simulink library "sm_trackV_lib_chain_track_s46"  (R2026a)
settings: Solver=VariableStepAuto
undefined symbols (not defined in the file): Excv, L1, L10, L11, L12, L13, L14, L15, L16, L17, L18, L19, L2, L20, L21, L22, L23, L24, L25, L26, L27, L28, L29, L3, L30, L31, L32, L33, L34, L35, L36, L37, L38, L39, L4, L40, L41, L42, L43, L44, L45, L46, L5, L6, L7, L8, L9, track_joint_targets
libraries: sm_trackV_lib_chain_segment x184
(part 5 of 5)

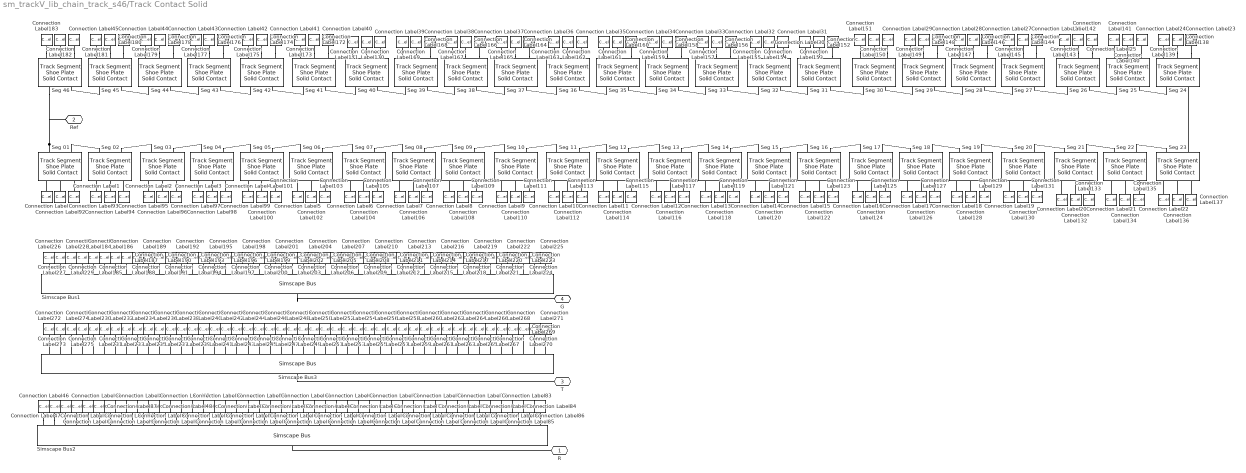
== system sm_trackV_lib_chain_track_s46/Track Contact Solid ==
  Connection Label : ConnectionLabel  Label=R1
  Connection Label1 : ConnectionLabel  Label=R2
  Connection Label10 : ConnectionLabel  Label=R11
  Connection Label100 : ConnectionLabel  Label=G5
  Connection Label101 : ConnectionLabel  Label=T5
  Connection Label102 : ConnectionLabel  Label=G6
  Connection Label103 : ConnectionLabel  Label=T6
  Connection Label104 : ConnectionLabel  Label=G7
  Connection Label105 : ConnectionLabel  Label=T7
  Connection Label106 : ConnectionLabel  Label=G8
  Connection Label107 : ConnectionLabel  Label=T8
  Connection Label108 : ConnectionLabel  Label=G9
  Connection Label109 : ConnectionLabel  Label=T9
  Connection Label11 : ConnectionLabel  Label=R12
  Connection Label110 : ConnectionLabel  Label=G10
  Connection Label111 : ConnectionLabel  Label=T10
  Connection Label112 : ConnectionLabel  Label=G11
  Connection Label113 : ConnectionLabel  Label=T11
  Connection Label114 : ConnectionLabel  Label=G12
  Connection Label115 : ConnectionLabel  Label=T12
  Connection Label116 : ConnectionLabel  Label=G13
  Connection Label117 : ConnectionLabel  Label=T13
  Connection Label118 : ConnectionLabel  Label=G14
  Connection Label119 : ConnectionLabel  Label=T14
  Connection Label12 : ConnectionLabel  Label=R13
  Connection Label120 : ConnectionLabel  Label=G15
  Connection Label121 : ConnectionLabel  Label=T15
  Connection Label122 : ConnectionLabel  Label=G16
  Connection Label123 : ConnectionLabel  Label=T16
  Connection Label124 : ConnectionLabel  Label=G17
  Connection Label125 : ConnectionLabel  Label=T17
  Connection Label126 : ConnectionLabel  Label=G18
  Connection Label127 : ConnectionLabel  Label=T18
  Connection Label128 : ConnectionLabel  Label=G19
  Connection Label129 : ConnectionLabel  Label=T19
  Connection Label13 : ConnectionLabel  Label=R14
  Connection Label130 : ConnectionLabel  Label=G20
  Connection Label131 : ConnectionLabel  Label=T20
  Connection Label132 : ConnectionLabel  Label=G21
  Connection Label133 : ConnectionLabel  Label=T21
  Connection Label134 : ConnectionLabel  Label=G22
  Connection Label135 : ConnectionLabel  Label=T22
  Connection Label136 : ConnectionLabel  Label=G23
  Connection Label137 : ConnectionLabel  Label=T23
  Connection Label138 : ConnectionLabel  Label=G24
  Connection Label139 : ConnectionLabel  Label=T24
  Connection Label14 : ConnectionLabel  Label=R15
  Connection Label140 : ConnectionLabel  Label=G25
  Connection Label141 : ConnectionLabel  Label=T25
  Connection Label142 : ConnectionLabel  Label=G26
  Connection Label143 : ConnectionLabel  Label=T26
  Connection Label144 : ConnectionLabel  Label=G27
  Connection Label145 : ConnectionLabel  Label=T27
  Connection Label146 : ConnectionLabel  Label=G28
  Connection Label147 : ConnectionLabel  Label=T28
  Connection Label148 : ConnectionLabel  Label=G29
  Connection Label149 : ConnectionLabel  Label=T29
  Connection Label15 : ConnectionLabel  Label=R16
  Connection Label150 : ConnectionLabel  Label=G30
  Connection Label151 : ConnectionLabel  Label=T30
  Connection Label152 : ConnectionLabel  Label=G31
  Connection Label153 : ConnectionLabel  Label=T31
  Connection Label154 : ConnectionLabel  Label=G32
  Connection Label155 : ConnectionLabel  Label=T32
  Connection Label156 : ConnectionLabel  Label=G33
  Connection Label157 : ConnectionLabel  Label=T33
  Connection Label158 : ConnectionLabel  Label=G34
  Connection Label159 : ConnectionLabel  Label=T34
  Connection Label16 : ConnectionLabel  Label=R17
  Connection Label160 : ConnectionLabel  Label=G35
  Connection Label161 : ConnectionLabel  Label=T35
  Connection Label162 : ConnectionLabel  Label=G36
  Connection Label163 : ConnectionLabel  Label=T36
  Connection Label164 : ConnectionLabel  Label=G37
  Connection Label165 : ConnectionLabel  Label=T37
  Connection Label166 : ConnectionLabel  Label=G38
  Connection Label167 : ConnectionLabel  Label=T38
  Connection Label168 : ConnectionLabel  Label=G39
  Connection Label169 : ConnectionLabel  Label=T39
  Connection Label17 : ConnectionLabel  Label=R18
  Connection Label170 : ConnectionLabel  Label=G40
  Connection Label171 : ConnectionLabel  Label=T40
  Connection Label172 : ConnectionLabel  Label=G41
  Connection Label173 : ConnectionLabel  Label=T41
  Connection Label174 : ConnectionLabel  Label=G42
  Connection Label175 : ConnectionLabel  Label=T42
  Connection Label176 : ConnectionLabel  Label=G43
  Connection Label177 : ConnectionLabel  Label=T43
  Connection Label178 : ConnectionLabel  Label=G44
  Connection Label179 : ConnectionLabel  Label=T44
  Connection Label18 : ConnectionLabel  Label=R19
  Connection Label180 : ConnectionLabel  Label=G45
  Connection Label181 : ConnectionLabel  Label=T45
  Connection Label182 : ConnectionLabel  Label=G46
  Connection Label183 : ConnectionLabel  Label=T46
  Connection Label184 : ConnectionLabel  Label=G5
  Connection Label185 : ConnectionLabel  Label=G6
  Connection Label186 : ConnectionLabel  Label=G7
  Connection Label187 : ConnectionLabel  Label=G8
  Connection Label188 : ConnectionLabel  Label=G9
  Connection Label189 : ConnectionLabel  Label=G10
  Connection Label19 : ConnectionLabel  Label=R20
  Connection Label190 : ConnectionLabel  Label=G11
  Connection Label191 : ConnectionLabel  Label=G12
  Connection Label192 : ConnectionLabel  Label=G13
  Connection Label193 : ConnectionLabel  Label=G14
  Connection Label194 : ConnectionLabel  Label=G15
  Connection Label195 : ConnectionLabel  Label=G16
  Connection Label196 : ConnectionLabel  Label=G17
  Connection Label197 : ConnectionLabel  Label=G18
  Connection Label198 : ConnectionLabel  Label=G19
  Connection Label199 : ConnectionLabel  Label=G20
  Connection Label2 : ConnectionLabel  Label=R3
  Connection Label20 : ConnectionLabel  Label=R21
  Connection Label200 : ConnectionLabel  Label=G21
  Connection Label201 : ConnectionLabel  Label=G22
  Connection Label202 : ConnectionLabel  Label=G23
  Connection Label203 : ConnectionLabel  Label=G24
  Connection Label204 : ConnectionLabel  Label=G25
  Connection Label205 : ConnectionLabel  Label=G26
  Connection Label206 : ConnectionLabel  Label=G27
  Connection Label207 : ConnectionLabel  Label=G28
  Connection Label208 : ConnectionLabel  Label=G29
  Connection Label209 : ConnectionLabel  Label=G30
  Connection Label21 : ConnectionLabel  Label=R22
  Connection Label210 : ConnectionLabel  Label=G31
  Connection Label211 : ConnectionLabel  Label=G32
  Connection Label212 : ConnectionLabel  Label=G33
  Connection Label213 : ConnectionLabel  Label=G34
  Connection Label214 : ConnectionLabel  Label=G35
  Connection Label215 : ConnectionLabel  Label=G36
  Connection Label216 : ConnectionLabel  Label=G37
  Connection Label217 : ConnectionLabel  Label=G38
  Connection Label218 : ConnectionLabel  Label=G39
  Connection Label219 : ConnectionLabel  Label=G40
  Connection Label22 : ConnectionLabel  Label=R23
  Connection Label220 : ConnectionLabel  Label=G41
  Connection Label221 : ConnectionLabel  Label=G42
  Connection Label222 : ConnectionLabel  Label=G43
  Connection Label223 : ConnectionLabel  Label=G44
  Connection Label224 : ConnectionLabel  Label=G45
  Connection Label225 : ConnectionLabel  Label=G46
  Connection Label226 : ConnectionLabel  Label=G1
  Connection Label227 : ConnectionLabel  Label=G2
  Connection Label228 : ConnectionLabel  Label=G3
  Connection Label229 : ConnectionLabel  Label=G4
  Connection Label23 : ConnectionLabel  Label=R24
  Connection Label230 : ConnectionLabel  Label=T5
  Connection Label231 : ConnectionLabel  Label=T6
  Connection Label232 : ConnectionLabel  Label=T7
  Connection Label233 : ConnectionLabel  Label=T8
  Connection Label234 : ConnectionLabel  Label=T9
  Connection Label235 : ConnectionLabel  Label=T10
  Connection Label236 : ConnectionLabel  Label=T11
  Connection Label237 : ConnectionLabel  Label=T12
  Connection Label238 : ConnectionLabel  Label=T13
  Connection Label239 : ConnectionLabel  Label=T14
  Connection Label24 : ConnectionLabel  Label=R25
  Connection Label240 : ConnectionLabel  Label=T15
  Connection Label241 : ConnectionLabel  Label=T16
  Connection Label242 : ConnectionLabel  Label=T17
  Connection Label243 : ConnectionLabel  Label=T18
  Connection Label244 : ConnectionLabel  Label=T19
  Connection Label245 : ConnectionLabel  Label=T20
  Connection Label246 : ConnectionLabel  Label=T21
  Connection Label247 : ConnectionLabel  Label=T22
  Connection Label248 : ConnectionLabel  Label=T23
  Connection Label249 : ConnectionLabel  Label=T24
  Connection Label25 : ConnectionLabel  Label=R26
  Connection Label250 : ConnectionLabel  Label=T25
  Connection Label251 : ConnectionLabel  Label=T26
  Connection Label252 : ConnectionLabel  Label=T27
  Connection Label253 : ConnectionLabel  Label=T28
  Connection Label254 : ConnectionLabel  Label=T29
  Connection Label255 : ConnectionLabel  Label=T30
  Connection Label256 : ConnectionLabel  Label=T31
  Connection Label257 : ConnectionLabel  Label=T32
  Connection Label258 : ConnectionLabel  Label=T33
  Connection Label259 : ConnectionLabel  Label=T34
  Connection Label26 : ConnectionLabel  Label=R27
  Connection Label260 : ConnectionLabel  Label=T35
  Connection Label261 : ConnectionLabel  Label=T36
  Connection Label262 : ConnectionLabel  Label=T37
  Connection Label263 : ConnectionLabel  Label=T38
  Connection Label264 : ConnectionLabel  Label=T39
  Connection Label265 : ConnectionLabel  Label=T40
  Connection Label266 : ConnectionLabel  Label=T41
  Connection Label267 : ConnectionLabel  Label=T42
  Connection Label268 : ConnectionLabel  Label=T43
  Connection Label269 : ConnectionLabel  Label=T44
  Connection Label27 : ConnectionLabel  Label=R28
  Connection Label270 : ConnectionLabel  Label=T45
  Connection Label271 : ConnectionLabel  Label=T46
  Connection Label272 : ConnectionLabel  Label=T1
  Connection Label273 : ConnectionLabel  Label=T2
  Connection Label274 : ConnectionLabel  Label=T3
  Connection Label275 : ConnectionLabel  Label=T4
  Connection Label28 : ConnectionLabel  Label=R29
  Connection Label29 : ConnectionLabel  Label=R30
  Connection Label3 : ConnectionLabel  Label=R4
  Connection Label30 : ConnectionLabel  Label=R31
  Connection Label31 : ConnectionLabel  Label=R32
  Connection Label32 : ConnectionLabel  Label=R33
  Connection Label33 : ConnectionLabel  Label=R34
  Connection Label34 : ConnectionLabel  Label=R35
  Connection Label35 : ConnectionLabel  Label=R36
  Connection Label36 : ConnectionLabel  Label=R37
  Connection Label37 : ConnectionLabel  Label=R38
  Connection Label38 : ConnectionLabel  Label=R39
  Connection Label39 : ConnectionLabel  Label=R40
  Connection Label4 : ConnectionLabel  Label=R5
  Connection Label40 : ConnectionLabel  Label=R41
  Connection Label41 : ConnectionLabel  Label=R42
  Connection Label42 : ConnectionLabel  Label=R43
  Connection Label43 : ConnectionLabel  Label=R44
  Connection Label44 : ConnectionLabel  Label=R45
  Connection Label45 : ConnectionLabel  Label=R46
  Connection Label46 : ConnectionLabel  Label=R1
  Connection Label47 : ConnectionLabel  Label=R2
  Connection Label48 : ConnectionLabel  Label=R11
  Connection Label49 : ConnectionLabel  Label=R12
  Connection Label5 : ConnectionLabel  Label=R6
  Connection Label50 : ConnectionLabel  Label=R13
  Connection Label51 : ConnectionLabel  Label=R14
  Connection Label52 : ConnectionLabel  Label=R15
  Connection Label53 : ConnectionLabel  Label=R16
  Connection Label54 : ConnectionLabel  Label=R17
  Connection Label55 : ConnectionLabel  Label=R18
  Connection Label56 : ConnectionLabel  Label=R19
  Connection Label57 : ConnectionLabel  Label=R20
  Connection Label58 : ConnectionLabel  Label=R3
  Connection Label59 : ConnectionLabel  Label=R21
  Connection Label6 : ConnectionLabel  Label=R7
  Connection Label60 : ConnectionLabel  Label=R22
  Connection Label61 : ConnectionLabel  Label=R23
  Connection Label62 : ConnectionLabel  Label=R24
  Connection Label63 : ConnectionLabel  Label=R25
  Connection Label64 : ConnectionLabel  Label=R26
  Connection Label65 : ConnectionLabel  Label=R27
  Connection Label66 : ConnectionLabel  Label=R28
  Connection Label67 : ConnectionLabel  Label=R29
  Connection Label68 : ConnectionLabel  Label=R30
  Connection Label69 : ConnectionLabel  Label=R4
  Connection Label7 : ConnectionLabel  Label=R8
  Connection Label70 : ConnectionLabel  Label=R31
  Connection Label71 : ConnectionLabel  Label=R32
  Connection Label72 : ConnectionLabel  Label=R33
  Connection Label73 : ConnectionLabel  Label=R34
  Connection Label74 : ConnectionLabel  Label=R35
  Connection Label75 : ConnectionLabel  Label=R36
  Connection Label76 : ConnectionLabel  Label=R37
  Connection Label77 : ConnectionLabel  Label=R38
  Connection Label78 : ConnectionLabel  Label=R39
  Connection Label79 : ConnectionLabel  Label=R40
  Connection Label8 : ConnectionLabel  Label=R9
  Connection Label80 : ConnectionLabel  Label=R5
  Connection Label81 : ConnectionLabel  Label=R41
  Connection Label82 : ConnectionLabel  Label=R42
  Connection Label83 : ConnectionLabel  Label=R43
  Connection Label84 : ConnectionLabel  Label=R44
  Connection Label85 : ConnectionLabel  Label=R45
  Connection Label86 : ConnectionLabel  Label=R46
  Connection Label87 : ConnectionLabel  Label=R6
  Connection Label88 : ConnectionLabel  Label=R7
  Connection Label89 : ConnectionLabel  Label=R8
  Connection Label9 : ConnectionLabel  Label=R10
  Connection Label90 : ConnectionLabel  Label=R9
  Connection Label91 : ConnectionLabel  Label=R10
  Connection Label92 : ConnectionLabel  Label=G1
  Connection Label93 : ConnectionLabel  Label=T1
  Connection Label94 : ConnectionLabel  Label=G2
  Connection Label95 : ConnectionLabel  Label=T2
  Connection Label96 : ConnectionLabel  Label=G3
  Connection Label97 : ConnectionLabel  Label=T3
  Connection Label98 : ConnectionLabel  Label=G4
  Connection Label99 : ConnectionLabel  Label=T4
  Seg 01 : sm_trackV_lib_chain_segment/Track Segment Shoe Plate Solid Contact  chain_wid=chain_wid  chain_seg_m=chain_seg_m  chain_seg_cg=chain_seg_cg  chain_seg_moi=chain_seg_moi  chain_seg_poi=chain_seg_poi  plate_h=plate_h  plate_xc=plate_xc  plate_thk=plate_thk  pin_sep=pin_sep  plate_ang=plate_ang  plate_clr=plate_clr  plate_opc=plate_opc  pin_len=pin_len  pin_rad=pin_rad  pin_clr=pin_clr  pin_opc=pin_opc  shoe_xc=shoe_xc  shoe_w=shoe_w  shoe_m=shoe_m  shoe_cg=shoe_cg  shoe_moi=shoe_moi  shoe_poi=shoe_poi  shoe_clr=shoe_clr  shoe_opc=shoe_opc  posTgtSpecify=on  posTgtPriority=Low  PositionTargetValue=32.8385  DampingCoefficient=chainDamping  shoe_plate_h=shoe_plate_h  shoe_plate_l=shoe_plate_l  shoe_plate_contact_clr=shoe_plate_contact_clr  shoe_plate_contact_opc=shoe_plate_contact_opc  chain_to_roller_clr=chain_to_roller_clr  chain_to_roller_opc=chain_to_roller_opc  chain_to_teeth_clr=chain_to_teeth_clr  chain_to_teeth_opc=chain_to_teeth_opc
      settings: LibrarySourceBlock=sm_chain_drive_lib/Link Shoe Points
  Seg 02 : sm_trackV_lib_chain_segment/Track Segment Shoe Plate Solid Contact  chain_wid=chain_wid  chain_seg_m=chain_seg_m  chain_seg_cg=chain_seg_cg  chain_seg_moi=chain_seg_moi  chain_seg_poi=chain_seg_poi  plate_h=plate_h  plate_xc=plate_xc  plate_thk=plate_thk  pin_sep=pin_sep  plate_ang=plate_ang  plate_clr=plate_clr  plate_opc=plate_opc  pin_len=pin_len  pin_rad=pin_rad  pin_clr=pin_clr  pin_opc=pin_opc  shoe_xc=shoe_xc  shoe_w=shoe_w  shoe_m=shoe_m  shoe_cg=shoe_cg  shoe_moi=shoe_moi  shoe_poi=shoe_poi  shoe_clr=shoe_clr  shoe_opc=shoe_opc  posTgtSpecify=on  posTgtPriority=Low  PositionTargetValue=32.8407  DampingCoefficient=chainDamping  shoe_plate_h=shoe_plate_h  shoe_plate_l=shoe_plate_l  shoe_plate_contact_clr=shoe_plate_contact_clr  shoe_plate_contact_opc=shoe_plate_contact_opc  chain_to_roller_clr=chain_to_roller_clr  chain_to_roller_opc=chain_to_roller_opc  chain_to_teeth_clr=chain_to_teeth_clr  chain_to_teeth_opc=chain_to_teeth_opc
      settings: LibrarySourceBlock=sm_chain_drive_lib/Tread Segment Shoe Plate Contact
  Seg 03 : sm_trackV_lib_chain_segment/Track Segment Shoe Plate Solid Contact  chain_wid=chain_wid  chain_seg_m=chain_seg_m  chain_seg_cg=chain_seg_cg  chain_seg_moi=chain_seg_moi  chain_seg_poi=chain_seg_poi  plate_h=plate_h  plate_xc=plate_xc  plate_thk=plate_thk  pin_sep=pin_sep  plate_ang=plate_ang  plate_clr=plate_clr  plate_opc=plate_opc  pin_len=pin_len  pin_rad=pin_rad  pin_clr=pin_clr  pin_opc=pin_opc  shoe_xc=shoe_xc  shoe_w=shoe_w  shoe_m=shoe_m  shoe_cg=shoe_cg  shoe_moi=shoe_moi  shoe_poi=shoe_poi  shoe_clr=shoe_clr  shoe_opc=shoe_opc  posTgtSpecify=on  posTgtPriority=Low  PositionTargetValue=32.6576  DampingCoefficient=chainDamping  shoe_plate_h=shoe_plate_h  shoe_plate_l=shoe_plate_l  shoe_plate_contact_clr=shoe_plate_contact_clr  shoe_plate_contact_opc=shoe_plate_contact_opc  chain_to_roller_clr=chain_to_roller_clr  chain_to_roller_opc=chain_to_roller_opc  chain_to_teeth_clr=chain_to_teeth_clr  chain_to_teeth_opc=chain_to_teeth_opc
      settings: LibrarySourceBlock=sm_chain_drive_lib/Tread Segment Shoe Plate Contact
  Seg 04 : sm_trackV_lib_chain_segment/Track Segment Shoe Plate Solid Contact  chain_wid=chain_wid  chain_seg_m=chain_seg_m  chain_seg_cg=chain_seg_cg  chain_seg_moi=chain_seg_moi  chain_seg_poi=chain_seg_poi  plate_h=plate_h  plate_xc=plate_xc  plate_thk=plate_thk  pin_sep=pin_sep  plate_ang=plate_ang  plate_clr=plate_clr  plate_opc=plate_opc  pin_len=pin_len  pin_rad=pin_rad  pin_clr=pin_clr  pin_opc=pin_opc  shoe_xc=shoe_xc  shoe_w=shoe_w  shoe_m=shoe_m  shoe_cg=shoe_cg  shoe_moi=shoe_moi  shoe_poi=shoe_poi  shoe_clr=shoe_clr  shoe_opc=shoe_opc  posTgtSpecify=on  posTgtPriority=Low  PositionTargetValue=5.447  DampingCoefficient=chainDamping  shoe_plate_h=shoe_plate_h  shoe_plate_l=shoe_plate_l  shoe_plate_contact_clr=shoe_plate_contact_clr  shoe_plate_contact_opc=shoe_plate_contact_opc  chain_to_roller_clr=chain_to_roller_clr  chain_to_roller_opc=chain_to_roller_opc  chain_to_teeth_clr=chain_to_teeth_clr  chain_to_teeth_opc=chain_to_teeth_opc
      settings: LibrarySourceBlock=sm_chain_drive_lib/Tread Segment Shoe Plate Contact
  Seg 05 : sm_trackV_lib_chain_segment/Track Segment Shoe Plate Solid Contact  chain_wid=chain_wid  chain_seg_m=chain_seg_m  chain_seg_cg=chain_seg_cg  chain_seg_moi=chain_seg_moi  chain_seg_poi=chain_seg_poi  plate_h=plate_h  plate_xc=plate_xc  plate_thk=plate_thk  pin_sep=pin_sep  plate_ang=plate_ang  plate_clr=plate_clr  plate_opc=plate_opc  pin_len=pin_len  pin_rad=pin_rad  pin_clr=pin_clr  pin_opc=pin_opc  shoe_xc=shoe_xc  shoe_w=shoe_w  shoe_m=shoe_m  shoe_cg=shoe_cg  shoe_moi=shoe_moi  shoe_poi=shoe_poi  shoe_clr=shoe_clr  shoe_opc=shoe_opc  posTgtSpecify=on  posTgtPriority=Low  PositionTargetValue=0.00013277  DampingCoefficient=chainDamping  shoe_plate_h=shoe_plate_h  shoe_plate_l=shoe_plate_l  shoe_plate_contact_clr=shoe_plate_contact_clr  shoe_plate_contact_opc=shoe_plate_contact_opc  chain_to_roller_clr=chain_to_roller_clr  chain_to_roller_opc=chain_to_roller_opc  chain_to_teeth_clr=chain_to_teeth_clr  chain_to_teeth_opc=chain_to_teeth_opc
      settings: LibrarySourceBlock=sm_chain_drive_lib/Tread Segment Shoe Plate Contact
  Seg 06 : sm_trackV_lib_chain_segment/Track Segment Shoe Plate Solid Contact  chain_wid=chain_wid  chain_seg_m=chain_seg_m  chain_seg_cg=chain_seg_cg  chain_seg_moi=chain_seg_moi  chain_seg_poi=chain_seg_poi  plate_h=plate_h  plate_xc=plate_xc  plate_thk=plate_thk  pin_sep=pin_sep  plate_ang=plate_ang  plate_clr=plate_clr  plate_opc=plate_opc  pin_len=pin_len  pin_rad=pin_rad  pin_clr=pin_clr  pin_opc=pin_opc  shoe_xc=shoe_xc  shoe_w=shoe_w  shoe_m=shoe_m  shoe_cg=shoe_cg  shoe_moi=shoe_moi  shoe_poi=shoe_poi  shoe_clr=shoe_clr  shoe_opc=shoe_opc  posTgtSpecify=on  posTgtPriority=Low  PositionTargetValue=1.7589  DampingCoefficient=chainDamping  shoe_plate_h=shoe_plate_h  shoe_plate_l=shoe_plate_l  shoe_plate_contact_clr=shoe_plate_contact_clr  shoe_plate_contact_opc=shoe_plate_contact_opc  chain_to_roller_clr=chain_to_roller_clr  chain_to_roller_opc=chain_to_roller_opc  chain_to_teeth_clr=chain_to_teeth_clr  chain_to_teeth_opc=chain_to_teeth_opc
      settings: LibrarySourceBlock=sm_chain_drive_lib/Tread Segment Shoe Plate Contact
  Seg 07 : sm_trackV_lib_chain_segment/Track Segment Shoe Plate Solid Contact  chain_wid=chain_wid  chain_seg_m=chain_seg_m  chain_seg_cg=chain_seg_cg  chain_seg_moi=chain_seg_moi  chain_seg_poi=chain_seg_poi  plate_h=plate_h  plate_xc=plate_xc  plate_thk=plate_thk  pin_sep=pin_sep  plate_ang=plate_ang  plate_clr=plate_clr  plate_opc=plate_opc  pin_len=pin_len  pin_rad=pin_rad  pin_clr=pin_clr  pin_opc=pin_opc  shoe_xc=shoe_xc  shoe_w=shoe_w  shoe_m=shoe_m  shoe_cg=shoe_cg  shoe_moi=shoe_moi  shoe_poi=shoe_poi  shoe_clr=shoe_clr  shoe_opc=shoe_opc  posTgtSpecify=on  posTgtPriority=Low  PositionTargetValue=0.86753  DampingCoefficient=chainDamping  shoe_plate_h=shoe_plate_h  shoe_plate_l=shoe_plate_l  shoe_plate_contact_clr=shoe_plate_contact_clr  shoe_plate_contact_opc=shoe_plate_contact_opc  chain_to_roller_clr=chain_to_roller_clr  chain_to_roller_opc=chain_to_roller_opc  chain_to_teeth_clr=chain_to_teeth_clr  chain_to_teeth_opc=chain_to_teeth_opc
      settings: LibrarySourceBlock=sm_chain_drive_lib/Tread Segment Shoe Plate Contact
  Seg 08 : sm_trackV_lib_chain_segment/Track Segment Shoe Plate Solid Contact  chain_wid=chain_wid  chain_seg_m=chain_seg_m  chain_seg_cg=chain_seg_cg  chain_seg_moi=chain_seg_moi  chain_seg_poi=chain_seg_poi  plate_h=plate_h  plate_xc=plate_xc  plate_thk=plate_thk  pin_sep=pin_sep  plate_ang=plate_ang  plate_clr=plate_clr  plate_opc=plate_opc  pin_len=pin_len  pin_rad=pin_rad  pin_clr=pin_clr  pin_opc=pin_opc  shoe_xc=shoe_xc  shoe_w=shoe_w  shoe_m=shoe_m  shoe_cg=shoe_cg  shoe_moi=shoe_moi  shoe_poi=shoe_poi  shoe_clr=shoe_clr  shoe_opc=shoe_opc  posTgtSpecify=on  posTgtPriority=Low  PositionTargetValue=-0.00014634  DampingCoefficient=chainDamping  shoe_plate_h=shoe_plate_h  shoe_plate_l=shoe_plate_l  shoe_plate_contact_clr=shoe_plate_contact_clr  shoe_plate_contact_opc=shoe_plate_contact_opc  chain_to_roller_clr=chain_to_roller_clr  chain_to_roller_opc=chain_to_roller_opc  chain_to_teeth_clr=chain_to_teeth_clr  chain_to_teeth_opc=chain_to_teeth_opc
      settings: LibrarySourceBlock=sm_chain_drive_lib/Tread Segment Shoe Plate Contact
  Seg 09 : sm_trackV_lib_chain_segment/Track Segment Shoe Plate Solid Contact  chain_wid=chain_wid  chain_seg_m=chain_seg_m  chain_seg_cg=chain_seg_cg  chain_seg_moi=chain_seg_moi  chain_seg_poi=chain_seg_poi  plate_h=plate_h  plate_xc=plate_xc  plate_thk=plate_thk  pin_sep=pin_sep  plate_ang=plate_ang  plate_clr=plate_clr  plate_opc=plate_opc  pin_len=pin_len  pin_rad=pin_rad  pin_clr=pin_clr  pin_opc=pin_opc  shoe_xc=shoe_xc  shoe_w=shoe_w  shoe_m=shoe_m  shoe_cg=shoe_cg  shoe_moi=shoe_moi  shoe_poi=shoe_poi  shoe_clr=shoe_clr  shoe_opc=shoe_opc  posTgtSpecify=on  posTgtPriority=Low  PositionTargetValue=-0.00033658  DampingCoefficient=chainDamping  shoe_plate_h=shoe_plate_h  shoe_plate_l=shoe_plate_l  shoe_plate_contact_clr=shoe_plate_contact_clr  shoe_plate_contact_opc=shoe_plate_contact_opc  chain_to_roller_clr=chain_to_roller_clr  chain_to_roller_opc=chain_to_roller_opc  chain_to_teeth_clr=chain_to_teeth_clr  chain_to_teeth_opc=chain_to_teeth_opc
      settings: LibrarySourceBlock=sm_chain_drive_lib/Tread Segment Shoe Plate Contact
  Seg 10 : sm_trackV_lib_chain_segment/Track Segment Shoe Plate Solid Contact  chain_wid=chain_wid  chain_seg_m=chain_seg_m  chain_seg_cg=chain_seg_cg  chain_seg_moi=chain_seg_moi  chain_seg_poi=chain_seg_poi  plate_h=plate_h  plate_xc=plate_xc  plate_thk=plate_thk  pin_sep=pin_sep  plate_ang=plate_ang  plate_clr=plate_clr  plate_opc=plate_opc  pin_len=pin_len  pin_rad=pin_rad  pin_clr=pin_clr  pin_opc=pin_opc  shoe_xc=shoe_xc  shoe_w=shoe_w  shoe_m=shoe_m  shoe_cg=shoe_cg  shoe_moi=shoe_moi  shoe_poi=shoe_poi  shoe_clr=shoe_clr  shoe_opc=shoe_opc  posTgtSpecify=on  posTgtPriority=Low  PositionTargetValue=-0.0004294  DampingCoefficient=chainDamping  shoe_plate_h=shoe_plate_h  shoe_plate_l=shoe_plate_l  shoe_plate_contact_clr=shoe_plate_contact_clr  shoe_plate_contact_opc=shoe_plate_contact_opc  chain_to_roller_clr=chain_to_roller_clr  chain_to_roller_opc=chain_to_roller_opc  chain_to_teeth_clr=chain_to_teeth_clr  chain_to_teeth_opc=chain_to_teeth_opc
      settings: LibrarySourceBlock=sm_chain_drive_lib/Tread Segment Shoe Plate Contact
  Seg 11 : sm_trackV_lib_chain_segment/Track Segment Shoe Plate Solid Contact  chain_wid=chain_wid  chain_seg_m=chain_seg_m  chain_seg_cg=chain_seg_cg  chain_seg_moi=chain_seg_moi  chain_seg_poi=chain_seg_poi  plate_h=plate_h  plate_xc=plate_xc  plate_thk=plate_thk  pin_sep=pin_sep  plate_ang=plate_ang  plate_clr=plate_clr  plate_opc=plate_opc  pin_len=pin_len  pin_rad=pin_rad  pin_clr=pin_clr  pin_opc=pin_opc  shoe_xc=shoe_xc  shoe_w=shoe_w  shoe_m=shoe_m  shoe_cg=shoe_cg  shoe_moi=shoe_moi  shoe_poi=shoe_poi  shoe_clr=shoe_clr  shoe_opc=shoe_opc  posTgtSpecify=on  posTgtPriority=Low  PositionTargetValue=-0.00049705  DampingCoefficient=chainDamping  shoe_plate_h=shoe_plate_h  shoe_plate_l=shoe_plate_l  shoe_plate_contact_clr=shoe_plate_contact_clr  shoe_plate_contact_opc=shoe_plate_contact_opc  chain_to_roller_clr=chain_to_roller_clr  chain_to_roller_opc=chain_to_roller_opc  chain_to_teeth_clr=chain_to_teeth_clr  chain_to_teeth_opc=chain_to_teeth_opc
      settings: LibrarySourceBlock=sm_chain_drive_lib/Tread Segment Shoe Plate Contact
  Seg 12 : sm_trackV_lib_chain_segment/Track Segment Shoe Plate Solid Contact  chain_wid=chain_wid  chain_seg_m=chain_seg_m  chain_seg_cg=chain_seg_cg  chain_seg_moi=chain_seg_moi  chain_seg_poi=chain_seg_poi  plate_h=plate_h  plate_xc=plate_xc  plate_thk=plate_thk  pin_sep=pin_sep  plate_ang=plate_ang  plate_clr=plate_clr  plate_opc=plate_opc  pin_len=pin_len  pin_rad=pin_rad  pin_clr=pin_clr  pin_opc=pin_opc  shoe_xc=shoe_xc  shoe_w=shoe_w  shoe_m=shoe_m  shoe_cg=shoe_cg  shoe_moi=shoe_moi  shoe_poi=shoe_poi  shoe_clr=shoe_clr  shoe_opc=shoe_opc  posTgtSpecify=on  posTgtPriority=Low  PositionTargetValue=-0.0005297  DampingCoefficient=chainDamping  shoe_plate_h=shoe_plate_h  shoe_plate_l=shoe_plate_l  shoe_plate_contact_clr=shoe_plate_contact_clr  shoe_plate_contact_opc=shoe_plate_contact_opc  chain_to_roller_clr=chain_to_roller_clr  chain_to_roller_opc=chain_to_roller_opc  chain_to_teeth_clr=chain_to_teeth_clr  chain_to_teeth_opc=chain_to_teeth_opc
      settings: LibrarySourceBlock=sm_chain_drive_lib/Tread Segment Shoe Plate Contact
  Seg 13 : sm_trackV_lib_chain_segment/Track Segment Shoe Plate Solid Contact  chain_wid=chain_wid  chain_seg_m=chain_seg_m  chain_seg_cg=chain_seg_cg  chain_seg_moi=chain_seg_moi  chain_seg_poi=chain_seg_poi  plate_h=plate_h  plate_xc=plate_xc  plate_thk=plate_thk  pin_sep=pin_sep  plate_ang=plate_ang  plate_clr=plate_clr  plate_opc=plate_opc  pin_len=pin_len  pin_rad=pin_rad  pin_clr=pin_clr  pin_opc=pin_opc  shoe_xc=shoe_xc  shoe_w=shoe_w  shoe_m=shoe_m  shoe_cg=shoe_cg  shoe_moi=shoe_moi  shoe_poi=shoe_poi  shoe_clr=shoe_clr  shoe_opc=shoe_opc  posTgtSpecify=on  posTgtPriority=Low  PositionTargetValue=-0.00052132  DampingCoefficient=chainDamping  shoe_plate_h=shoe_plate_h  shoe_plate_l=shoe_plate_l  shoe_plate_contact_clr=shoe_plate_contact_clr  shoe_plate_contact_opc=shoe_plate_contact_opc  chain_to_roller_clr=chain_to_roller_clr  chain_to_roller_opc=chain_to_roller_opc  chain_to_teeth_clr=chain_to_teeth_clr  chain_to_teeth_opc=chain_to_teeth_opc
      settings: LibrarySourceBlock=sm_chain_drive_lib/Tread Segment Shoe Plate Contact
  Seg 14 : sm_trackV_lib_chain_segment/Track Segment Shoe Plate Solid Contact  chain_wid=chain_wid  chain_seg_m=chain_seg_m  chain_seg_cg=chain_seg_cg  chain_seg_moi=chain_seg_moi  chain_seg_poi=chain_seg_poi  plate_h=plate_h  plate_xc=plate_xc  plate_thk=plate_thk  pin_sep=pin_sep  plate_ang=plate_ang  plate_clr=plate_clr  plate_opc=plate_opc  pin_len=pin_len  pin_rad=pin_rad  pin_clr=pin_clr  pin_opc=pin_opc  shoe_xc=shoe_xc  shoe_w=shoe_w  shoe_m=shoe_m  shoe_cg=shoe_cg  shoe_moi=shoe_moi  shoe_poi=shoe_poi  shoe_clr=shoe_clr  shoe_opc=shoe_opc  posTgtSpecify=on  posTgtPriority=Low  PositionTargetValue=-0.00046966  DampingCoefficient=chainDamping  shoe_plate_h=shoe_plate_h  shoe_plate_l=shoe_plate_l  shoe_plate_contact_clr=shoe_plate_contact_clr  shoe_plate_contact_opc=shoe_plate_contact_opc  chain_to_roller_clr=chain_to_roller_clr  chain_to_roller_opc=chain_to_roller_opc  chain_to_teeth_clr=chain_to_teeth_clr  chain_to_teeth_opc=chain_to_teeth_opc
      settings: LibrarySourceBlock=sm_chain_drive_lib/Tread Segment Shoe Plate Contact
  Seg 15 : sm_trackV_lib_chain_segment/Track Segment Shoe Plate Solid Contact  chain_wid=chain_wid  chain_seg_m=chain_seg_m  chain_seg_cg=chain_seg_cg  chain_seg_moi=chain_seg_moi  chain_seg_poi=chain_seg_poi  plate_h=plate_h  plate_xc=plate_xc  plate_thk=plate_thk  pin_sep=pin_sep  plate_ang=plate_ang  plate_clr=plate_clr  plate_opc=plate_opc  pin_len=pin_len  pin_rad=pin_rad  pin_clr=pin_clr  pin_opc=pin_opc  shoe_xc=shoe_xc  shoe_w=shoe_w  shoe_m=shoe_m  shoe_cg=shoe_cg  shoe_moi=shoe_moi  shoe_poi=shoe_poi  shoe_clr=shoe_clr  shoe_opc=shoe_opc  posTgtSpecify=on  posTgtPriority=Low  PositionTargetValue=-0.00038011  DampingCoefficient=chainDamping  shoe_plate_h=shoe_plate_h  shoe_plate_l=shoe_plate_l  shoe_plate_contact_clr=shoe_plate_contact_clr  shoe_plate_contact_opc=shoe_plate_contact_opc  chain_to_roller_clr=chain_to_roller_clr  chain_to_roller_opc=chain_to_roller_opc  chain_to_teeth_clr=chain_to_teeth_clr  chain_to_teeth_opc=chain_to_teeth_opc
      settings: LibrarySourceBlock=sm_chain_drive_lib/Tread Segment Shoe Plate Contact
  Seg 16 : sm_trackV_lib_chain_segment/Track Segment Shoe Plate Solid Contact  chain_wid=chain_wid  chain_seg_m=chain_seg_m  chain_seg_cg=chain_seg_cg  chain_seg_moi=chain_seg_moi  chain_seg_poi=chain_seg_poi  plate_h=plate_h  plate_xc=plate_xc  plate_thk=plate_thk  pin_sep=pin_sep  plate_ang=plate_ang  plate_clr=plate_clr  plate_opc=plate_opc  pin_len=pin_len  pin_rad=pin_rad  pin_clr=pin_clr  pin_opc=pin_opc  shoe_xc=shoe_xc  shoe_w=shoe_w  shoe_m=shoe_m  shoe_cg=shoe_cg  shoe_moi=shoe_moi  shoe_poi=shoe_poi  shoe_clr=shoe_clr  shoe_opc=shoe_opc  posTgtSpecify=on  posTgtPriority=Low  PositionTargetValue=-0.00026621  DampingCoefficient=chainDamping  shoe_plate_h=shoe_plate_h  shoe_plate_l=shoe_plate_l  shoe_plate_contact_clr=shoe_plate_contact_clr  shoe_plate_contact_opc=shoe_plate_contact_opc  chain_to_roller_clr=chain_to_roller_clr  chain_to_roller_opc=chain_to_roller_opc  chain_to_teeth_clr=chain_to_teeth_clr  chain_to_teeth_opc=chain_to_teeth_opc
      settings: LibrarySourceBlock=sm_chain_drive_lib/Tread Segment Shoe Plate Contact
  Seg 17 : sm_trackV_lib_chain_segment/Track Segment Shoe Plate Solid Contact  chain_wid=chain_wid  chain_seg_m=chain_seg_m  chain_seg_cg=chain_seg_cg  chain_seg_moi=chain_seg_moi  chain_seg_poi=chain_seg_poi  plate_h=plate_h  plate_xc=plate_xc  plate_thk=plate_thk  pin_sep=pin_sep  plate_ang=plate_ang  plate_clr=plate_clr  plate_opc=plate_opc  pin_len=pin_len  pin_rad=pin_rad  pin_clr=pin_clr  pin_opc=pin_opc  shoe_xc=shoe_xc  shoe_w=shoe_w  shoe_m=shoe_m  shoe_cg=shoe_cg  shoe_moi=shoe_moi  shoe_poi=shoe_poi  shoe_clr=shoe_clr  shoe_opc=shoe_opc  posTgtSpecify=on  posTgtPriority=Low  PositionTargetValue=4.6763e-05  DampingCoefficient=chainDamping  shoe_plate_h=shoe_plate_h  shoe_plate_l=shoe_plate_l  shoe_plate_contact_clr=shoe_plate_contact_clr  shoe_plate_contact_opc=shoe_plate_contact_opc  chain_to_roller_clr=chain_to_roller_clr  chain_to_roller_opc=chain_to_roller_opc  chain_to_teeth_clr=chain_to_teeth_clr  chain_to_teeth_opc=chain_to_teeth_opc
      settings: LibrarySourceBlock=sm_chain_drive_lib/Tread Segment Shoe Plate Contact
  Seg 18 : sm_trackV_lib_chain_segment/Track Segment Shoe Plate Solid Contact  chain_wid=chain_wid  chain_seg_m=chain_seg_m  chain_seg_cg=chain_seg_cg  chain_seg_moi=chain_seg_moi  chain_seg_poi=chain_seg_poi  plate_h=plate_h  plate_xc=plate_xc  plate_thk=plate_thk  pin_sep=pin_sep  plate_ang=plate_ang  plate_clr=plate_clr  plate_opc=plate_opc  pin_len=pin_len  pin_rad=pin_rad  pin_clr=pin_clr  pin_opc=pin_opc  shoe_xc=shoe_xc  shoe_w=shoe_w  shoe_m=shoe_m  shoe_cg=shoe_cg  shoe_moi=shoe_moi  shoe_poi=shoe_poi  shoe_clr=shoe_clr  shoe_opc=shoe_opc  posTgtSpecify=on  posTgtPriority=Low  PositionTargetValue=1.1075  DampingCoefficient=chainDamping  shoe_plate_h=shoe_plate_h  shoe_plate_l=shoe_plate_l  shoe_plate_contact_clr=shoe_plate_contact_clr  shoe_plate_contact_opc=shoe_plate_contact_opc  chain_to_roller_clr=chain_to_roller_clr  chain_to_roller_opc=chain_to_roller_opc  chain_to_teeth_clr=chain_to_teeth_clr  chain_to_teeth_opc=chain_to_teeth_opc
      settings: LibrarySourceBlock=sm_chain_drive_lib/Tread Segment Shoe Plate Contact
  Seg 19 : sm_trackV_lib_chain_segment/Track Segment Shoe Plate Solid Contact  chain_wid=chain_wid  chain_seg_m=chain_seg_m  chain_seg_cg=chain_seg_cg  chain_seg_moi=chain_seg_moi  chain_seg_poi=chain_seg_poi  plate_h=plate_h  plate_xc=plate_xc  plate_thk=plate_thk  pin_sep=pin_sep  plate_ang=plate_ang  plate_clr=plate_clr  plate_opc=plate_opc  pin_len=pin_len  pin_rad=pin_rad  pin_clr=pin_clr  pin_opc=pin_opc  shoe_xc=shoe_xc  shoe_w=shoe_w  shoe_m=shoe_m  shoe_cg=shoe_cg  shoe_moi=shoe_moi  shoe_poi=shoe_poi  shoe_clr=shoe_clr  shoe_opc=shoe_opc  posTgtSpecify=on  posTgtPriority=Low  PositionTargetValue=0.12453  DampingCoefficient=chainDamping  shoe_plate_h=shoe_plate_h  shoe_plate_l=shoe_plate_l  shoe_plate_contact_clr=shoe_plate_contact_clr  shoe_plate_contact_opc=shoe_plate_contact_opc  chain_to_roller_clr=chain_to_roller_clr  chain_to_roller_opc=chain_to_roller_opc  chain_to_teeth_clr=chain_to_teeth_clr  chain_to_teeth_opc=chain_to_teeth_opc
      settings: LibrarySourceBlock=sm_chain_drive_lib/Tread Segment Shoe Plate Contact
  Seg 20 : sm_trackV_lib_chain_segment/Track Segment Shoe Plate Solid Contact  chain_wid=chain_wid  chain_seg_m=chain_seg_m  chain_seg_cg=chain_seg_cg  chain_seg_moi=chain_seg_moi  chain_seg_poi=chain_seg_poi  plate_h=plate_h  plate_xc=plate_xc  plate_thk=plate_thk  pin_sep=pin_sep  plate_ang=plate_ang  plate_clr=plate_clr  plate_opc=plate_opc  pin_len=pin_len  pin_rad=pin_rad  pin_clr=pin_clr  pin_opc=pin_opc  shoe_xc=shoe_xc  shoe_w=shoe_w  shoe_m=shoe_m  shoe_cg=shoe_cg  shoe_moi=shoe_moi  shoe_poi=shoe_poi  shoe_clr=shoe_clr  shoe_opc=shoe_opc  posTgtSpecify=on  posTgtPriority=Low  PositionTargetValue=6.4867e-05  DampingCoefficient=chainDamping  shoe_plate_h=shoe_plate_h  shoe_plate_l=shoe_plate_l  shoe_plate_contact_clr=shoe_plate_contact_clr  shoe_plate_contact_opc=shoe_plate_contact_opc  chain_to_roller_clr=chain_to_roller_clr  chain_to_roller_opc=chain_to_roller_opc  chain_to_teeth_clr=chain_to_teeth_clr  chain_to_teeth_opc=chain_to_teeth_opc
      settings: LibrarySourceBlock=sm_chain_drive_lib/Tread Segment Shoe Plate Contact
  Seg 21 : sm_trackV_lib_chain_segment/Track Segment Shoe Plate Solid Contact  chain_wid=chain_wid  chain_seg_m=chain_seg_m  chain_seg_cg=chain_seg_cg  chain_seg_moi=chain_seg_moi  chain_seg_poi=chain_seg_poi  plate_h=plate_h  plate_xc=plate_xc  plate_thk=plate_thk  pin_sep=pin_sep  plate_ang=plate_ang  plate_clr=plate_clr  plate_opc=plate_opc  pin_len=pin_len  pin_rad=pin_rad  pin_clr=pin_clr  pin_opc=pin_opc  shoe_xc=shoe_xc  shoe_w=shoe_w  shoe_m=shoe_m  shoe_cg=shoe_cg  shoe_moi=shoe_moi  shoe_poi=shoe_poi  shoe_clr=shoe_clr  shoe_opc=shoe_opc  posTgtSpecify=on  posTgtPriority=Low  PositionTargetValue=11.1152  DampingCoefficient=chainDamping  shoe_plate_h=shoe_plate_h  shoe_plate_l=shoe_plate_l  shoe_plate_contact_clr=shoe_plate_contact_clr  shoe_plate_contact_opc=shoe_plate_contact_opc  chain_to_roller_clr=chain_to_roller_clr  chain_to_roller_opc=chain_to_roller_opc  chain_to_teeth_clr=chain_to_teeth_clr  chain_to_teeth_opc=chain_to_teeth_opc
      settings: LibrarySourceBlock=sm_chain_drive_lib/Tread Segment Shoe Plate Contact
  Seg 22 : sm_trackV_lib_chain_segment/Track Segment Shoe Plate Solid Contact  chain_wid=chain_wid  chain_seg_m=chain_seg_m  chain_seg_cg=chain_seg_cg  chain_seg_moi=chain_seg_moi  chain_seg_poi=chain_seg_poi  plate_h=plate_h  plate_xc=plate_xc  plate_thk=plate_thk  pin_sep=pin_sep  plate_ang=plate_ang  plate_clr=plate_clr  plate_opc=plate_opc  pin_len=pin_len  pin_rad=pin_rad  pin_clr=pin_clr  pin_opc=pin_opc  shoe_xc=shoe_xc  shoe_w=shoe_w  shoe_m=shoe_m  shoe_cg=shoe_cg  shoe_moi=shoe_moi  shoe_poi=shoe_poi  shoe_clr=shoe_clr  shoe_opc=shoe_opc  posTgtSpecify=on  posTgtPriority=Low  PositionTargetValue=30.3431  DampingCoefficient=chainDamping  shoe_plate_h=shoe_plate_h  shoe_plate_l=shoe_plate_l  shoe_plate_contact_clr=shoe_plate_contact_clr  shoe_plate_contact_opc=shoe_plate_contact_opc  chain_to_roller_clr=chain_to_roller_clr  chain_to_roller_opc=chain_to_roller_opc  chain_to_teeth_clr=chain_to_teeth_clr  chain_to_teeth_opc=chain_to_teeth_opc
      settings: LibrarySourceBlock=sm_chain_drive_lib/Tread Segment Shoe Plate Contact
  Seg 23 : sm_trackV_lib_chain_segment/Track Segment Shoe Plate Solid Contact  chain_wid=chain_wid  chain_seg_m=chain_seg_m  chain_seg_cg=chain_seg_cg  chain_seg_moi=chain_seg_moi  chain_seg_poi=chain_seg_poi  plate_h=plate_h  plate_xc=plate_xc  plate_thk=plate_thk  pin_sep=pin_sep  plate_ang=plate_ang  plate_clr=plate_clr  plate_opc=plate_opc  pin_len=pin_len  pin_rad=pin_rad  pin_clr=pin_clr  pin_opc=pin_opc  shoe_xc=shoe_xc  shoe_w=shoe_w  shoe_m=shoe_m  shoe_cg=shoe_cg  shoe_moi=shoe_moi  shoe_poi=shoe_poi  shoe_clr=shoe_clr  shoe_opc=shoe_opc  posTgtSpecify=on  posTgtPriority=Low  PositionTargetValue=32.3566  DampingCoefficient=chainDamping  shoe_plate_h=shoe_plate_h  shoe_plate_l=shoe_plate_l  shoe_plate_contact_clr=shoe_plate_contact_clr  shoe_plate_contact_opc=shoe_plate_contact_opc  chain_to_roller_clr=chain_to_roller_clr  chain_to_roller_opc=chain_to_roller_opc  chain_to_teeth_clr=chain_to_teeth_clr  chain_to_teeth_opc=chain_to_teeth_opc
      settings: LibrarySourceBlock=sm_chain_drive_lib/Tread Segment Shoe Plate Contact
  Seg 24 : sm_trackV_lib_chain_segment/Track Segment Shoe Plate Solid Contact  chain_wid=chain_wid  chain_seg_m=chain_seg_m  chain_seg_cg=chain_seg_cg  chain_seg_moi=chain_seg_moi  chain_seg_poi=chain_seg_poi  plate_h=plate_h  plate_xc=plate_xc  plate_thk=plate_thk  pin_sep=pin_sep  plate_ang=plate_ang  plate_clr=plate_clr  plate_opc=plate_opc  pin_len=pin_len  pin_rad=pin_rad  pin_clr=pin_clr  pin_opc=pin_opc  shoe_xc=shoe_xc  shoe_w=shoe_w  shoe_m=shoe_m  shoe_cg=shoe_cg  shoe_moi=shoe_moi  shoe_poi=shoe_poi  shoe_clr=shoe_clr  shoe_opc=shoe_opc  posTgtSpecify=on  posTgtPriority=Low  PositionTargetValue=31.2315  DampingCoefficient=chainDamping  shoe_plate_h=shoe_plate_h  shoe_plate_l=shoe_plate_l  shoe_plate_contact_clr=shoe_plate_contact_clr  shoe_plate_contact_opc=shoe_plate_contact_opc  chain_to_roller_clr=chain_to_roller_clr  chain_to_roller_opc=chain_to_roller_opc  chain_to_teeth_clr=chain_to_teeth_clr  chain_to_teeth_opc=chain_to_teeth_opc
      settings: LibrarySourceBlock=sm_chain_drive_lib/Tread Segment Shoe Plate Contact
  Seg 25 : sm_trackV_lib_chain_segment/Track Segment Shoe Plate Solid Contact  chain_wid=chain_wid  chain_seg_m=chain_seg_m  chain_seg_cg=chain_seg_cg  chain_seg_moi=chain_seg_moi  chain_seg_poi=chain_seg_poi  plate_h=plate_h  plate_xc=plate_xc  plate_thk=plate_thk  pin_sep=pin_sep  plate_ang=plate_ang  plate_clr=plate_clr  plate_opc=plate_opc  pin_len=pin_len  pin_rad=pin_rad  pin_clr=pin_clr  pin_opc=pin_opc  shoe_xc=shoe_xc  shoe_w=shoe_w  shoe_m=shoe_m  shoe_cg=shoe_cg  shoe_moi=shoe_moi  shoe_poi=shoe_poi  shoe_clr=shoe_clr  shoe_opc=shoe_opc  posTgtSpecify=on  posTgtPriority=Low  PositionTargetValue=32.7074  DampingCoefficient=chainDamping  shoe_plate_h=shoe_plate_h  shoe_plate_l=shoe_plate_l  shoe_plate_contact_clr=shoe_plate_contact_clr  shoe_plate_contact_opc=shoe_plate_contact_opc  chain_to_roller_clr=chain_to_roller_clr  chain_to_roller_opc=chain_to_roller_opc  chain_to_teeth_clr=chain_to_teeth_clr  chain_to_teeth_opc=chain_to_teeth_opc
      settings: LibrarySourceBlock=sm_chain_drive_lib/Tread Segment Shoe Plate Contact
  Seg 26 : sm_trackV_lib_chain_segment/Track Segment Shoe Plate Solid Contact  chain_wid=chain_wid  chain_seg_m=chain_seg_m  chain_seg_cg=chain_seg_cg  chain_seg_moi=chain_seg_moi  chain_seg_poi=chain_seg_poi  plate_h=plate_h  plate_xc=plate_xc  plate_thk=plate_thk  pin_sep=pin_sep  plate_ang=plate_ang  plate_clr=plate_clr  plate_opc=plate_opc  pin_len=pin_len  pin_rad=pin_rad  pin_clr=pin_clr  pin_opc=pin_opc  shoe_xc=shoe_xc  shoe_w=shoe_w  shoe_m=shoe_m  shoe_cg=shoe_cg  shoe_moi=shoe_moi  shoe_poi=shoe_poi  shoe_clr=shoe_clr  shoe_opc=shoe_opc  posTgtSpecify=on  posTgtPriority=Low  PositionTargetValue=29.2112  DampingCoefficient=chainDamping  shoe_plate_h=shoe_plate_h  shoe_plate_l=shoe_plate_l  shoe_plate_contact_clr=shoe_plate_contact_clr  shoe_plate_contact_opc=shoe_plate_contact_opc  chain_to_roller_clr=chain_to_roller_clr  chain_to_roller_opc=chain_to_roller_opc  chain_to_teeth_clr=chain_to_teeth_clr  chain_to_teeth_opc=chain_to_teeth_opc
      settings: LibrarySourceBlock=sm_chain_drive_lib/Tread Segment Shoe Plate Contact
  Seg 27 : sm_trackV_lib_chain_segment/Track Segment Shoe Plate Solid Contact  chain_wid=chain_wid  chain_seg_m=chain_seg_m  chain_seg_cg=chain_seg_cg  chain_seg_moi=chain_seg_moi  chain_seg_poi=chain_seg_poi  plate_h=plate_h  plate_xc=plate_xc  plate_thk=plate_thk  pin_sep=pin_sep  plate_ang=plate_ang  plate_clr=plate_clr  plate_opc=plate_opc  pin_len=pin_len  pin_rad=pin_rad  pin_clr=pin_clr  pin_opc=pin_opc  shoe_xc=shoe_xc  shoe_w=shoe_w  shoe_m=shoe_m  shoe_cg=shoe_cg  shoe_moi=shoe_moi  shoe_poi=shoe_poi  shoe_clr=shoe_clr  shoe_opc=shoe_opc  posTgtSpecify=on  posTgtPriority=Low  PositionTargetValue=7.6812  DampingCoefficient=chainDamping  shoe_plate_h=shoe_plate_h  shoe_plate_l=shoe_plate_l  shoe_plate_contact_clr=shoe_plate_contact_clr  shoe_plate_contact_opc=shoe_plate_contact_opc  chain_to_roller_clr=chain_to_roller_clr  chain_to_roller_opc=chain_to_roller_opc  chain_to_teeth_clr=chain_to_teeth_clr  chain_to_teeth_opc=chain_to_teeth_opc
      settings: LibrarySourceBlock=sm_chain_drive_lib/Tread Segment Shoe Plate Contact
  Seg 28 : sm_trackV_lib_chain_segment/Track Segment Shoe Plate Solid Contact  chain_wid=chain_wid  chain_seg_m=chain_seg_m  chain_seg_cg=chain_seg_cg  chain_seg_moi=chain_seg_moi  chain_seg_poi=chain_seg_poi  plate_h=plate_h  plate_xc=plate_xc  plate_thk=plate_thk  pin_sep=pin_sep  plate_ang=plate_ang  plate_clr=plate_clr  plate_opc=plate_opc  pin_len=pin_len  pin_rad=pin_rad  pin_clr=pin_clr  pin_opc=pin_opc  shoe_xc=shoe_xc  shoe_w=shoe_w  shoe_m=shoe_m  shoe_cg=shoe_cg  shoe_moi=shoe_moi  shoe_poi=shoe_poi  shoe_clr=shoe_clr  shoe_opc=shoe_opc  posTgtSpecify=on  posTgtPriority=Low  PositionTargetValue=-3.9493e-05  DampingCoefficient=chainDamping  shoe_plate_h=shoe_plate_h  shoe_plate_l=shoe_plate_l  shoe_plate_contact_clr=shoe_plate_contact_clr  shoe_plate_contact_opc=shoe_plate_contact_opc  chain_to_roller_clr=chain_to_roller_clr  chain_to_roller_opc=chain_to_roller_opc  chain_to_teeth_clr=chain_to_teeth_clr  chain_to_teeth_opc=chain_to_teeth_opc
      settings: LibrarySourceBlock=sm_chain_drive_lib/Tread Segment Shoe Plate Contact
  Seg 29 : sm_trackV_lib_chain_segment/Track Segment Shoe Plate Solid Contact  chain_wid=chain_wid  chain_seg_m=chain_seg_m  chain_seg_cg=chain_seg_cg  chain_seg_moi=chain_seg_moi  chain_seg_poi=chain_seg_poi  plate_h=plate_h  plate_xc=plate_xc  plate_thk=plate_thk  pin_sep=pin_sep  plate_ang=plate_ang  plate_clr=plate_clr  plate_opc=plate_opc  pin_len=pin_len  pin_rad=pin_rad  pin_clr=pin_clr  pin_opc=pin_opc  shoe_xc=shoe_xc  shoe_w=shoe_w  shoe_m=shoe_m  shoe_cg=shoe_cg  shoe_moi=shoe_moi  shoe_poi=shoe_poi  shoe_clr=shoe_clr  shoe_opc=shoe_opc  posTgtSpecify=on  posTgtPriority=Low  PositionTargetValue=-4.2189e-05  DampingCoefficient=chainDamping  shoe_plate_h=shoe_plate_h  shoe_plate_l=shoe_plate_l  shoe_plate_contact_clr=shoe_plate_contact_clr  shoe_plate_contact_opc=shoe_plate_contact_opc  chain_to_roller_clr=chain_to_roller_clr  chain_to_roller_opc=chain_to_roller_opc  chain_to_teeth_clr=chain_to_teeth_clr  chain_to_teeth_opc=chain_to_teeth_opc
      settings: LibrarySourceBlock=sm_chain_drive_lib/Tread Segment Shoe Plate Contact
  Seg 30 : sm_trackV_lib_chain_segment/Track Segment Shoe Plate Solid Contact  chain_wid=chain_wid  chain_seg_m=chain_seg_m  chain_seg_cg=chain_seg_cg  chain_seg_moi=chain_seg_moi  chain_seg_poi=chain_seg_poi  plate_h=plate_h  plate_xc=plate_xc  plate_thk=plate_thk  pin_sep=pin_sep  plate_ang=plate_ang  plate_clr=plate_clr  plate_opc=plate_opc  pin_len=pin_len  pin_rad=pin_rad  pin_clr=pin_clr  pin_opc=pin_opc  shoe_xc=shoe_xc  shoe_w=shoe_w  shoe_m=shoe_m  shoe_cg=shoe_cg  shoe_moi=shoe_moi  shoe_poi=shoe_poi  shoe_clr=shoe_clr  shoe_opc=shoe_opc  posTgtSpecify=on  posTgtPriority=Low  PositionTargetValue=-3.4821e-05  DampingCoefficient=chainDamping  shoe_plate_h=shoe_plate_h  shoe_plate_l=shoe_plate_l  shoe_plate_contact_clr=shoe_plate_contact_clr  shoe_plate_contact_opc=shoe_plate_contact_opc  chain_to_roller_clr=chain_to_roller_clr  chain_to_roller_opc=chain_to_roller_opc  chain_to_teeth_clr=chain_to_teeth_clr  chain_to_teeth_opc=chain_to_teeth_opc
      settings: LibrarySourceBlock=sm_chain_drive_lib/Tread Segment Shoe Plate Contact
  Seg 31 : sm_trackV_lib_chain_segment/Track Segment Shoe Plate Solid Contact  chain_wid=chain_wid  chain_seg_m=chain_seg_m  chain_seg_cg=chain_seg_cg  chain_seg_moi=chain_seg_moi  chain_seg_poi=chain_seg_poi  plate_h=plate_h  plate_xc=plate_xc  plate_thk=plate_thk  pin_sep=pin_sep  plate_ang=plate_ang  plate_clr=plate_clr  plate_opc=plate_opc  pin_len=pin_len  pin_rad=pin_rad  pin_clr=pin_clr  pin_opc=pin_opc  shoe_xc=shoe_xc  shoe_w=shoe_w  shoe_m=shoe_m  shoe_cg=shoe_cg  shoe_moi=shoe_moi  shoe_poi=shoe_poi  shoe_clr=shoe_clr  shoe_opc=shoe_opc  posTgtSpecify=on  posTgtPriority=Low  PositionTargetValue=-3.2281e-05  DampingCoefficient=chainDamping  shoe_plate_h=shoe_plate_h  shoe_plate_l=shoe_plate_l  shoe_plate_contact_clr=shoe_plate_contact_clr  shoe_plate_contact_opc=shoe_plate_contact_opc  chain_to_roller_clr=chain_to_roller_clr  chain_to_roller_opc=chain_to_roller_opc  chain_to_teeth_clr=chain_to_teeth_clr  chain_to_teeth_opc=chain_to_teeth_opc
      settings: LibrarySourceBlock=sm_chain_drive_lib/Tread Segment Shoe Plate Contact
  Seg 32 : sm_trackV_lib_chain_segment/Track Segment Shoe Plate Solid Contact  chain_wid=chain_wid  chain_seg_m=chain_seg_m  chain_seg_cg=chain_seg_cg  chain_seg_moi=chain_seg_moi  chain_seg_poi=chain_seg_poi  plate_h=plate_h  plate_xc=plate_xc  plate_thk=plate_thk  pin_sep=pin_sep  plate_ang=plate_ang  plate_clr=plate_clr  plate_opc=plate_opc  pin_len=pin_len  pin_rad=pin_rad  pin_clr=pin_clr  pin_opc=pin_opc  shoe_xc=shoe_xc  shoe_w=shoe_w  shoe_m=shoe_m  shoe_cg=shoe_cg  shoe_moi=shoe_moi  shoe_poi=shoe_poi  shoe_clr=shoe_clr  shoe_opc=shoe_opc  posTgtSpecify=on  posTgtPriority=Low  PositionTargetValue=-2.2438e-05  DampingCoefficient=chainDamping  shoe_plate_h=shoe_plate_h  shoe_plate_l=shoe_plate_l  shoe_plate_contact_clr=shoe_plate_contact_clr  shoe_plate_contact_opc=shoe_plate_contact_opc  chain_to_roller_clr=chain_to_roller_clr  chain_to_roller_opc=chain_to_roller_opc  chain_to_teeth_clr=chain_to_teeth_clr  chain_to_teeth_opc=chain_to_teeth_opc
      settings: LibrarySourceBlock=sm_chain_drive_lib/Tread Segment Shoe Plate Contact
  Seg 33 : sm_trackV_lib_chain_segment/Track Segment Shoe Plate Solid Contact  chain_wid=chain_wid  chain_seg_m=chain_seg_m  chain_seg_cg=chain_seg_cg  chain_seg_moi=chain_seg_moi  chain_seg_poi=chain_seg_poi  plate_h=plate_h  plate_xc=plate_xc  plate_thk=plate_thk  pin_sep=pin_sep  plate_ang=plate_ang  plate_clr=plate_clr  plate_opc=plate_opc  pin_len=pin_len  pin_rad=pin_rad  pin_clr=pin_clr  pin_opc=pin_opc  shoe_xc=shoe_xc  shoe_w=shoe_w  shoe_m=shoe_m  shoe_cg=shoe_cg  shoe_moi=shoe_moi  shoe_poi=shoe_poi  shoe_clr=shoe_clr  shoe_opc=shoe_opc  posTgtSpecify=on  posTgtPriority=Low  PositionTargetValue=3.4114  DampingCoefficient=chainDamping  shoe_plate_h=shoe_plate_h  shoe_plate_l=shoe_plate_l  shoe_plate_contact_clr=shoe_plate_contact_clr  shoe_plate_contact_opc=shoe_plate_contact_opc  chain_to_roller_clr=chain_to_roller_clr  chain_to_roller_opc=chain_to_roller_opc  chain_to_teeth_clr=chain_to_teeth_clr  chain_to_teeth_opc=chain_to_teeth_opc
      settings: LibrarySourceBlock=sm_chain_drive_lib/Tread Segment Shoe Plate Contact
  Seg 34 : sm_trackV_lib_chain_segment/Track Segment Shoe Plate Solid Contact  chain_wid=chain_wid  chain_seg_m=chain_seg_m  chain_seg_cg=chain_seg_cg  chain_seg_moi=chain_seg_moi  chain_seg_poi=chain_seg_poi  plate_h=plate_h  plate_xc=plate_xc  plate_thk=plate_thk  pin_sep=pin_sep  plate_ang=plate_ang  plate_clr=plate_clr  plate_opc=plate_opc  pin_len=pin_len  pin_rad=pin_rad  pin_clr=pin_clr  pin_opc=pin_opc  shoe_xc=shoe_xc  shoe_w=shoe_w  shoe_m=shoe_m  shoe_cg=shoe_cg  shoe_moi=shoe_moi  shoe_poi=shoe_poi  shoe_clr=shoe_clr  shoe_opc=shoe_opc  posTgtSpecify=on  posTgtPriority=Low  PositionTargetValue=0.47561  DampingCoefficient=chainDamping  shoe_plate_h=shoe_plate_h  shoe_plate_l=shoe_plate_l  shoe_plate_contact_clr=shoe_plate_contact_clr  shoe_plate_contact_opc=shoe_plate_contact_opc  chain_to_roller_clr=chain_to_roller_clr  chain_to_roller_opc=chain_to_roller_opc  chain_to_teeth_clr=chain_to_teeth_clr  chain_to_teeth_opc=chain_to_teeth_opc
      settings: LibrarySourceBlock=sm_chain_drive_lib/Tread Segment Shoe Plate Contact
  Seg 35 : sm_trackV_lib_chain_segment/Track Segment Shoe Plate Solid Contact  chain_wid=chain_wid  chain_seg_m=chain_seg_m  chain_seg_cg=chain_seg_cg  chain_seg_moi=chain_seg_moi  chain_seg_poi=chain_seg_poi  plate_h=plate_h  plate_xc=plate_xc  plate_thk=plate_thk  pin_sep=pin_sep  plate_ang=plate_ang  plate_clr=plate_clr  plate_opc=plate_opc  pin_len=pin_len  pin_rad=pin_rad  pin_clr=pin_clr  pin_opc=pin_opc  shoe_xc=shoe_xc  shoe_w=shoe_w  shoe_m=shoe_m  shoe_cg=shoe_cg  shoe_moi=shoe_moi  shoe_poi=shoe_poi  shoe_clr=shoe_clr  shoe_opc=shoe_opc  posTgtSpecify=on  posTgtPriority=Low  PositionTargetValue=-1.2501e-05  DampingCoefficient=chainDamping  shoe_plate_h=shoe_plate_h  shoe_plate_l=shoe_plate_l  shoe_plate_contact_clr=shoe_plate_contact_clr  shoe_plate_contact_opc=shoe_plate_contact_opc  chain_to_roller_clr=chain_to_roller_clr  chain_to_roller_opc=chain_to_roller_opc  chain_to_teeth_clr=chain_to_teeth_clr  chain_to_teeth_opc=chain_to_teeth_opc
      settings: LibrarySourceBlock=sm_chain_drive_lib/Tread Segment Shoe Plate Contact
  Seg 36 : sm_trackV_lib_chain_segment/Track Segment Shoe Plate Solid Contact  chain_wid=chain_wid  chain_seg_m=chain_seg_m  chain_seg_cg=chain_seg_cg  chain_seg_moi=chain_seg_moi  chain_seg_poi=chain_seg_poi  plate_h=plate_h  plate_xc=plate_xc  plate_thk=plate_thk  pin_sep=pin_sep  plate_ang=plate_ang  plate_clr=plate_clr  plate_opc=plate_opc  pin_len=pin_len  pin_rad=pin_rad  pin_clr=pin_clr  pin_opc=pin_opc  shoe_xc=shoe_xc  shoe_w=shoe_w  shoe_m=shoe_m  shoe_cg=shoe_cg  shoe_moi=shoe_moi  shoe_poi=shoe_poi  shoe_clr=shoe_clr  shoe_opc=shoe_opc  posTgtSpecify=on  posTgtPriority=Low  PositionTargetValue=-7.1543e-06  DampingCoefficient=chainDamping  shoe_plate_h=shoe_plate_h  shoe_plate_l=shoe_plate_l  shoe_plate_contact_clr=shoe_plate_contact_clr  shoe_plate_contact_opc=shoe_plate_contact_opc  chain_to_roller_clr=chain_to_roller_clr  chain_to_roller_opc=chain_to_roller_opc  chain_to_teeth_clr=chain_to_teeth_clr  chain_to_teeth_opc=chain_to_teeth_opc
      settings: LibrarySourceBlock=sm_chain_drive_lib/Tread Segment Shoe Plate Contact
  Seg 37 : sm_trackV_lib_chain_segment/Track Segment Shoe Plate Solid Contact  chain_wid=chain_wid  chain_seg_m=chain_seg_m  chain_seg_cg=chain_seg_cg  chain_seg_moi=chain_seg_moi  chain_seg_poi=chain_seg_poi  plate_h=plate_h  plate_xc=plate_xc  plate_thk=plate_thk  pin_sep=pin_sep  plate_ang=plate_ang  plate_clr=plate_clr  plate_opc=plate_opc  pin_len=pin_len  pin_rad=pin_rad  pin_clr=pin_clr  pin_opc=pin_opc  shoe_xc=shoe_xc  shoe_w=shoe_w  shoe_m=shoe_m  shoe_cg=shoe_cg  shoe_moi=shoe_moi  shoe_poi=shoe_poi  shoe_clr=shoe_clr  shoe_opc=shoe_opc  posTgtSpecify=on  posTgtPriority=Low  PositionTargetValue=-3.1816e-06  DampingCoefficient=chainDamping  shoe_plate_h=shoe_plate_h  shoe_plate_l=shoe_plate_l  shoe_plate_contact_clr=shoe_plate_contact_clr  shoe_plate_contact_opc=shoe_plate_contact_opc  chain_to_roller_clr=chain_to_roller_clr  chain_to_roller_opc=chain_to_roller_opc  chain_to_teeth_clr=chain_to_teeth_clr  chain_to_teeth_opc=chain_to_teeth_opc
      settings: LibrarySourceBlock=sm_chain_drive_lib/Tread Segment Shoe Plate Contact
  Seg 38 : sm_trackV_lib_chain_segment/Track Segment Shoe Plate Solid Contact  chain_wid=chain_wid  chain_seg_m=chain_seg_m  chain_seg_cg=chain_seg_cg  chain_seg_moi=chain_seg_moi  chain_seg_poi=chain_seg_poi  plate_h=plate_h  plate_xc=plate_xc  plate_thk=plate_thk  pin_sep=pin_sep  plate_ang=plate_ang  plate_clr=plate_clr  plate_opc=plate_opc  pin_len=pin_len  pin_rad=pin_rad  pin_clr=pin_clr  pin_opc=pin_opc  shoe_xc=shoe_xc  shoe_w=shoe_w  shoe_m=shoe_m  shoe_cg=shoe_cg  shoe_moi=shoe_moi  shoe_poi=shoe_poi  shoe_clr=shoe_clr  shoe_opc=shoe_opc  posTgtSpecify=on  posTgtPriority=Low  PositionTargetValue=3.4032  DampingCoefficient=chainDamping  shoe_plate_h=shoe_plate_h  shoe_plate_l=shoe_plate_l  shoe_plate_contact_clr=shoe_plate_contact_clr  shoe_plate_contact_opc=shoe_plate_contact_opc  chain_to_roller_clr=chain_to_roller_clr  chain_to_roller_opc=chain_to_roller_opc  chain_to_teeth_clr=chain_to_teeth_clr  chain_to_teeth_opc=chain_to_teeth_opc
      settings: LibrarySourceBlock=sm_chain_drive_lib/Tread Segment Shoe Plate Contact
  Seg 39 : sm_trackV_lib_chain_segment/Track Segment Shoe Plate Solid Contact  chain_wid=chain_wid  chain_seg_m=chain_seg_m  chain_seg_cg=chain_seg_cg  chain_seg_moi=chain_seg_moi  chain_seg_poi=chain_seg_poi  plate_h=plate_h  plate_xc=plate_xc  plate_thk=plate_thk  pin_sep=pin_sep  plate_ang=plate_ang  plate_clr=plate_clr  plate_opc=plate_opc  pin_len=pin_len  pin_rad=pin_rad  pin_clr=pin_clr  pin_opc=pin_opc  shoe_xc=shoe_xc  shoe_w=shoe_w  shoe_m=shoe_m  shoe_cg=shoe_cg  shoe_moi=shoe_moi  shoe_poi=shoe_poi  shoe_clr=shoe_clr  shoe_opc=shoe_opc  posTgtSpecify=on  posTgtPriority=Low  PositionTargetValue=2.9598  DampingCoefficient=chainDamping  shoe_plate_h=shoe_plate_h  shoe_plate_l=shoe_plate_l  shoe_plate_contact_clr=shoe_plate_contact_clr  shoe_plate_contact_opc=shoe_plate_contact_opc  chain_to_roller_clr=chain_to_roller_clr  chain_to_roller_opc=chain_to_roller_opc  chain_to_teeth_clr=chain_to_teeth_clr  chain_to_teeth_opc=chain_to_teeth_opc
      settings: LibrarySourceBlock=sm_chain_drive_lib/Tread Segment Shoe Plate Contact
  Seg 40 : sm_trackV_lib_chain_segment/Track Segment Shoe Plate Solid Contact  chain_wid=chain_wid  chain_seg_m=chain_seg_m  chain_seg_cg=chain_seg_cg  chain_seg_moi=chain_seg_moi  chain_seg_poi=chain_seg_poi  plate_h=plate_h  plate_xc=plate_xc  plate_thk=plate_thk  pin_sep=pin_sep  plate_ang=plate_ang  plate_clr=plate_clr  plate_opc=plate_opc  pin_len=pin_len  pin_rad=pin_rad  pin_clr=pin_clr  pin_opc=pin_opc  shoe_xc=shoe_xc  shoe_w=shoe_w  shoe_m=shoe_m  shoe_cg=shoe_cg  shoe_moi=shoe_moi  shoe_poi=shoe_poi  shoe_clr=shoe_clr  shoe_opc=shoe_opc  posTgtSpecify=on  posTgtPriority=Low  PositionTargetValue=-2.8638e-06  DampingCoefficient=chainDamping  shoe_plate_h=shoe_plate_h  shoe_plate_l=shoe_plate_l  shoe_plate_contact_clr=shoe_plate_contact_clr  shoe_plate_contact_opc=shoe_plate_contact_opc  chain_to_roller_clr=chain_to_roller_clr  chain_to_roller_opc=chain_to_roller_opc  chain_to_teeth_clr=chain_to_teeth_clr  chain_to_teeth_opc=chain_to_teeth_opc
      settings: LibrarySourceBlock=sm_chain_drive_lib/Tread Segment Shoe Plate Contact
  Seg 41 : sm_trackV_lib_chain_segment/Track Segment Shoe Plate Solid Contact  chain_wid=chain_wid  chain_seg_m=chain_seg_m  chain_seg_cg=chain_seg_cg  chain_seg_moi=chain_seg_moi  chain_seg_poi=chain_seg_poi  plate_h=plate_h  plate_xc=plate_xc  plate_thk=plate_thk  pin_sep=pin_sep  plate_ang=plate_ang  plate_clr=plate_clr  plate_opc=plate_opc  pin_len=pin_len  pin_rad=pin_rad  pin_clr=pin_clr  pin_opc=pin_opc  shoe_xc=shoe_xc  shoe_w=shoe_w  shoe_m=shoe_m  shoe_cg=shoe_cg  shoe_moi=shoe_moi  shoe_poi=shoe_poi  shoe_clr=shoe_clr  shoe_opc=shoe_opc  posTgtSpecify=on  posTgtPriority=Low  PositionTargetValue=-2.2795e-06  DampingCoefficient=chainDamping  shoe_plate_h=shoe_plate_h  shoe_plate_l=shoe_plate_l  shoe_plate_contact_clr=shoe_plate_contact_clr  shoe_plate_contact_opc=shoe_plate_contact_opc  chain_to_roller_clr=chain_to_roller_clr  chain_to_roller_opc=chain_to_roller_opc  chain_to_teeth_clr=chain_to_teeth_clr  chain_to_teeth_opc=chain_to_teeth_opc
      settings: LibrarySourceBlock=sm_chain_drive_lib/Tread Segment Shoe Plate Contact
  Seg 42 : sm_trackV_lib_chain_segment/Track Segment Shoe Plate Solid Contact  chain_wid=chain_wid  chain_seg_m=chain_seg_m  chain_seg_cg=chain_seg_cg  chain_seg_moi=chain_seg_moi  chain_seg_poi=chain_seg_poi  plate_h=plate_h  plate_xc=plate_xc  plate_thk=plate_thk  pin_sep=pin_sep  plate_ang=plate_ang  plate_clr=plate_clr  plate_opc=plate_opc  pin_len=pin_len  pin_rad=pin_rad  pin_clr=pin_clr  pin_opc=pin_opc  shoe_xc=shoe_xc  shoe_w=shoe_w  shoe_m=shoe_m  shoe_cg=shoe_cg  shoe_moi=shoe_moi  shoe_poi=shoe_poi  shoe_clr=shoe_clr  shoe_opc=shoe_opc  posTgtSpecify=off  posTgtPriority=Low  PositionTargetValue=1.1558e-07  DampingCoefficient=chainDamping  shoe_plate_h=shoe_plate_h  shoe_plate_l=shoe_plate_l  shoe_plate_contact_clr=shoe_plate_contact_clr  shoe_plate_contact_opc=shoe_plate_contact_opc  chain_to_roller_clr=chain_to_roller_clr  chain_to_roller_opc=chain_to_roller_opc  chain_to_teeth_clr=chain_to_teeth_clr  chain_to_teeth_opc=chain_to_teeth_opc
      settings: LibrarySourceBlock=sm_chain_drive_lib/Tread Segment Shoe Plate Contact
  Seg 43 : sm_trackV_lib_chain_segment/Track Segment Shoe Plate Solid Contact  chain_wid=chain_wid  chain_seg_m=chain_seg_m  chain_seg_cg=chain_seg_cg  chain_seg_moi=chain_seg_moi  chain_seg_poi=chain_seg_poi  plate_h=plate_h  plate_xc=plate_xc  plate_thk=plate_thk  pin_sep=pin_sep  plate_ang=plate_ang  plate_clr=plate_clr  plate_opc=plate_opc  pin_len=pin_len  pin_rad=pin_rad  pin_clr=pin_clr  pin_opc=pin_opc  shoe_xc=shoe_xc  shoe_w=shoe_w  shoe_m=shoe_m  shoe_cg=shoe_cg  shoe_moi=shoe_moi  shoe_poi=shoe_poi  shoe_clr=shoe_clr  shoe_opc=shoe_opc  posTgtSpecify=on  posTgtPriority=Low  PositionTargetValue=-1.1779e-06  DampingCoefficient=chainDamping  shoe_plate_h=shoe_plate_h  shoe_plate_l=shoe_plate_l  shoe_plate_contact_clr=shoe_plate_contact_clr  shoe_plate_contact_opc=shoe_plate_contact_opc  chain_to_roller_clr=chain_to_roller_clr  chain_to_roller_opc=chain_to_roller_opc  chain_to_teeth_clr=chain_to_teeth_clr  chain_to_teeth_opc=chain_to_teeth_opc
      settings: LibrarySourceBlock=sm_chain_drive_lib/Tread Segment Shoe Plate Contact
  Seg 44 : sm_trackV_lib_chain_segment/Track Segment Shoe Plate Solid Contact  chain_wid=chain_wid  chain_seg_m=chain_seg_m  chain_seg_cg=chain_seg_cg  chain_seg_moi=chain_seg_moi  chain_seg_poi=chain_seg_poi  plate_h=plate_h  plate_xc=plate_xc  plate_thk=plate_thk  pin_sep=pin_sep  plate_ang=plate_ang  plate_clr=plate_clr  plate_opc=plate_opc  pin_len=pin_len  pin_rad=pin_rad  pin_clr=pin_clr  pin_opc=pin_opc  shoe_xc=shoe_xc  shoe_w=shoe_w  shoe_m=shoe_m  shoe_cg=shoe_cg  shoe_moi=shoe_moi  shoe_poi=shoe_poi  shoe_clr=shoe_clr  shoe_opc=shoe_opc  posTgtSpecify=on  posTgtPriority=Low  PositionTargetValue=2.0157  DampingCoefficient=chainDamping  shoe_plate_h=shoe_plate_h  shoe_plate_l=shoe_plate_l  shoe_plate_contact_clr=shoe_plate_contact_clr  shoe_plate_contact_opc=shoe_plate_contact_opc  chain_to_roller_clr=chain_to_roller_clr  chain_to_roller_opc=chain_to_roller_opc  chain_to_teeth_clr=chain_to_teeth_clr  chain_to_teeth_opc=chain_to_teeth_opc
      settings: LibrarySourceBlock=sm_chain_drive_lib/Tread Segment Shoe Plate Contact
  Seg 45 : sm_trackV_lib_chain_segment/Track Segment Shoe Plate Solid Contact  chain_wid=chain_wid  chain_seg_m=chain_seg_m  chain_seg_cg=chain_seg_cg  chain_seg_moi=chain_seg_moi  chain_seg_poi=chain_seg_poi  plate_h=plate_h  plate_xc=plate_xc  plate_thk=plate_thk  pin_sep=pin_sep  plate_ang=plate_ang  plate_clr=plate_clr  plate_opc=plate_opc  pin_len=pin_len  pin_rad=pin_rad  pin_clr=pin_clr  pin_opc=pin_opc  shoe_xc=shoe_xc  shoe_w=shoe_w  shoe_m=shoe_m  shoe_cg=shoe_cg  shoe_moi=shoe_moi  shoe_poi=shoe_poi  shoe_clr=shoe_clr  shoe_opc=shoe_opc  posTgtSpecify=on  posTgtPriority=Low  PositionTargetValue=32.612  DampingCoefficient=chainDamping  shoe_plate_h=shoe_plate_h  shoe_plate_l=shoe_plate_l  shoe_plate_contact_clr=shoe_plate_contact_clr  shoe_plate_contact_opc=shoe_plate_contact_opc  chain_to_roller_clr=chain_to_roller_clr  chain_to_roller_opc=chain_to_roller_opc  chain_to_teeth_clr=chain_to_teeth_clr  chain_to_teeth_opc=chain_to_teeth_opc
      settings: LibrarySourceBlock=sm_chain_drive_lib/Tread Segment Shoe Plate Contact
  Seg 46 : sm_trackV_lib_chain_segment/Track Segment Shoe Plate Solid Contact  chain_wid=chain_wid  chain_seg_m=chain_seg_m  chain_seg_cg=chain_seg_cg  chain_seg_moi=chain_seg_moi  chain_seg_poi=chain_seg_poi  plate_h=plate_h  plate_xc=plate_xc  plate_thk=plate_thk  pin_sep=pin_sep  plate_ang=plate_ang  plate_clr=plate_clr  plate_opc=plate_opc  pin_len=pin_len  pin_rad=pin_rad  pin_clr=pin_clr  pin_opc=pin_opc  shoe_xc=shoe_xc  shoe_w=shoe_w  shoe_m=shoe_m  shoe_cg=shoe_cg  shoe_moi=shoe_moi  shoe_poi=shoe_poi  shoe_clr=shoe_clr  shoe_opc=shoe_opc  posTgtSpecify=on  posTgtPriority=Low  PositionTargetValue=32.8373  DampingCoefficient=chainDamping  shoe_plate_h=shoe_plate_h  shoe_plate_l=shoe_plate_l  shoe_plate_contact_clr=shoe_plate_contact_clr  shoe_plate_contact_opc=shoe_plate_contact_opc  chain_to_roller_clr=chain_to_roller_clr  chain_to_roller_opc=chain_to_roller_opc  chain_to_teeth_clr=chain_to_teeth_clr  chain_to_teeth_opc=chain_to_teeth_opc
      settings: LibrarySourceBlock=sm_chain_drive_lib/Tread Segment Shoe Plate Contact
  Simscape Bus1 : SimscapeBus  HierarchyStrings=L1;L2;L3;L4;L5;L6;L7;L8;L9;L10;L11;L12;L13;L14;L15;L16;L17;L18;L19;L20;L21;L22;L23;L24;L25;L26;L27;L28;L29;L30;L31;L32;L33;L34;L35;L36;L37;L38;L39;L40;L41;L42;L43;L44;L45;L46  ConnectionType=Bus: CBO_Chain46
  Simscape Bus2 : SimscapeBus  HierarchyStrings=L1;L2;L3;L4;L5;L6;L7;L8;L9;L10;L11;L12;L13;L14;L15;L16;L17;L18;L19;L20;L21;L22;L23;L24;L25;L26;L27;L28;L29;L30;L31;L32;L33;L34;L35;L36;L37;L38;L39;L40;L41;L42;L43;L44;L45;L46  ConnectionType=Bus: CBO_Chain46
  Simscape Bus3 : SimscapeBus  HierarchyStrings=L1;L2;L3;L4;L5;L6;L7;L8;L9;L10;L11;L12;L13;L14;L15;L16;L17;L18;L19;L20;L21;L22;L23;L24;L25;L26;L27;L28;L29;L30;L31;L32;L33;L34;L35;L36;L37;L38;L39;L40;L41;L42;L43;L44;L45;L46  ConnectionType=Bus: CBO_Chain46
  R : PMIOPort  Side=Left
  Ref : PMIOPort  Port=2  Side=Left
  T : PMIOPort  Port=3  Side=Left
  G : PMIOPort  Port=4  Side=Right
  connections:
  Seg 01/LConn1 -- Seg 46/LConn2 -- Ref/RConn1
  Seg 45/LConn2 -- Seg 46/LConn1
  Seg 44/LConn2 -- Seg 45/LConn1
  Seg 43/LConn2 -- Seg 44/LConn1
  Seg 42/LConn2 -- Seg 43/LConn1
  Seg 41/LConn2 -- Seg 42/LConn1
  Seg 40/LConn2 -- Seg 41/LConn1
  Seg 39/LConn2 -- Seg 40/LConn1
  Seg 38/LConn2 -- Seg 39/LConn1
  Seg 37/LConn2 -- Seg 38/LConn1
  Seg 36/LConn2 -- Seg 37/LConn1
  Seg 35/LConn2 -- Seg 36/LConn1
  Seg 34/LConn2 -- Seg 35/LConn1
  Seg 33/LConn2 -- Seg 34/LConn1
  Seg 32/LConn2 -- Seg 33/LConn1
  Seg 31/LConn2 -- Seg 32/LConn1
  Seg 30/LConn2 -- Seg 31/LConn1
  Seg 29/LConn2 -- Seg 30/LConn1
  Seg 28/LConn2 -- Seg 29/LConn1
  Seg 27/LConn2 -- Seg 28/LConn1
  Seg 26/LConn2 -- Seg 27/LConn1
  Seg 25/LConn2 -- Seg 26/LConn1
  Seg 24/LConn2 -- Seg 25/LConn1
  Seg 23/LConn2 -- Seg 24/LConn1
  Seg 22/LConn2 -- Seg 23/LConn1
  Seg 21/LConn2 -- Seg 22/LConn1
  Seg 20/LConn2 -- Seg 21/LConn1
  Seg 19/LConn2 -- Seg 20/LConn1
  Seg 18/LConn2 -- Seg 19/LConn1
  Seg 17/LConn2 -- Seg 18/LConn1
  Seg 17/LConn1 -- Seg 16/LConn2
  Seg 16/LConn1 -- Seg 15/LConn2
  Seg 15/LConn1 -- Seg 14/LConn2
  Seg 14/LConn1 -- Seg 13/LConn2
  Seg 13/LConn1 -- Seg 12/LConn2
  Seg 12/LConn1 -- Seg 11/LConn2
  Seg 11/LConn1 -- Seg 10/LConn2
  Seg 10/LConn1 -- Seg 09/LConn2
  Seg 09/LConn1 -- Seg 08/LConn2
  Seg 08/LConn1 -- Seg 07/LConn2
  Seg 07/LConn1 -- Seg 06/LConn2
  Seg 06/LConn1 -- Seg 05/LConn2
  Seg 05/LConn1 -- Seg 04/LConn2
  Seg 04/LConn1 -- Seg 03/LConn2
  Seg 03/LConn1 -- Seg 02/LConn2
  Seg 01/LConn2 -- Seg 02/LConn1
  Connection Label183/LConn1 -- Seg 46/RConn3
  Connection Label182/LConn1 -- Seg 46/RConn2
  Connection Label45/LConn1 -- Seg 46/RConn1
  Connection Label181/LConn1 -- Seg 45/RConn3
  Connection Label180/LConn1 -- Seg 45/RConn2
  Connection Label44/LConn1 -- Seg 45/RConn1
  Connection Label179/LConn1 -- Seg 44/RConn3
  Connection Label178/LConn1 -- Seg 44/RConn2
  Connection Label43/LConn1 -- Seg 44/RConn1
  Connection Label177/LConn1 -- Seg 43/RConn3
  Connection Label176/LConn1 -- Seg 43/RConn2
  Connection Label42/LConn1 -- Seg 43/RConn1
  Connection Label175/LConn1 -- Seg 42/RConn3
  Connection Label174/LConn1 -- Seg 42/RConn2
  Connection Label41/LConn1 -- Seg 42/RConn1
  Connection Label173/LConn1 -- Seg 41/RConn3
  Connection Label172/LConn1 -- Seg 41/RConn2
  Connection Label40/LConn1 -- Seg 41/RConn1
  Connection Label171/LConn1 -- Seg 40/RConn3
  Connection Label170/LConn1 -- Seg 40/RConn2
  Connection Label39/LConn1 -- Seg 40/RConn1
  Connection Label169/LConn1 -- Seg 39/RConn3
  Connection Label168/LConn1 -- Seg 39/RConn2
  Connection Label38/LConn1 -- Seg 39/RConn1
  Connection Label167/LConn1 -- Seg 38/RConn3
  Connection Label166/LConn1 -- Seg 38/RConn2
  Connection Label37/LConn1 -- Seg 38/RConn1
  Connection Label165/LConn1 -- Seg 37/RConn3
  Connection Label164/LConn1 -- Seg 37/RConn2
  Connection Label36/LConn1 -- Seg 37/RConn1
  Connection Label163/LConn1 -- Seg 36/RConn3
  Connection Label162/LConn1 -- Seg 36/RConn2
  Connection Label35/LConn1 -- Seg 36/RConn1
  Connection Label161/LConn1 -- Seg 35/RConn3
  Connection Label160/LConn1 -- Seg 35/RConn2
  Connection Label34/LConn1 -- Seg 35/RConn1
  Connection Label159/LConn1 -- Seg 34/RConn3
  Connection Label158/LConn1 -- Seg 34/RConn2
  Connection Label33/LConn1 -- Seg 34/RConn1
  Connection Label157/LConn1 -- Seg 33/RConn3
  Connection Label156/LConn1 -- Seg 33/RConn2
  Connection Label32/LConn1 -- Seg 33/RConn1
  Connection Label155/LConn1 -- Seg 32/RConn3
  Connection Label154/LConn1 -- Seg 32/RConn2
  Connection Label31/LConn1 -- Seg 32/RConn1
  Connection Label153/LConn1 -- Seg 31/RConn3
  Connection Label152/LConn1 -- Seg 31/RConn2
  Connection Label30/LConn1 -- Seg 31/RConn1
  Connection Label151/LConn1 -- Seg 30/RConn3
  Connection Label150/LConn1 -- Seg 30/RConn2
  Connection Label29/LConn1 -- Seg 30/RConn1
  Connection Label149/LConn1 -- Seg 29/RConn3
  Connection Label148/LConn1 -- Seg 29/RConn2
  Connection Label28/LConn1 -- Seg 29/RConn1
  Connection Label147/LConn1 -- Seg 28/RConn3
  Connection Label146/LConn1 -- Seg 28/RConn2
  Connection Label27/LConn1 -- Seg 28/RConn1
  Connection Label145/LConn1 -- Seg 27/RConn3
  Connection Label144/LConn1 -- Seg 27/RConn2
  Connection Label26/LConn1 -- Seg 27/RConn1
  Connection Label143/LConn1 -- Seg 26/RConn3
  Connection Label142/LConn1 -- Seg 26/RConn2
  Connection Label25/LConn1 -- Seg 26/RConn1
  Connection Label141/LConn1 -- Seg 25/RConn3
  Connection Label140/LConn1 -- Seg 25/RConn2
  Connection Label24/LConn1 -- Seg 25/RConn1
  Connection Label139/LConn1 -- Seg 24/RConn3
  Connection Label138/LConn1 -- Seg 24/RConn2
  Connection Label23/LConn1 -- Seg 24/RConn1
  Connection Label137/LConn1 -- Seg 23/RConn3
  Connection Label136/LConn1 -- Seg 23/RConn2
  Connection Label22/LConn1 -- Seg 23/RConn1
  Connection Label135/LConn1 -- Seg 22/RConn3
  Connection Label134/LConn1 -- Seg 22/RConn2
  Connection Label21/LConn1 -- Seg 22/RConn1
  Connection Label133/LConn1 -- Seg 21/RConn3
  Connection Label132/LConn1 -- Seg 21/RConn2
  Connection Label20/LConn1 -- Seg 21/RConn1
  Connection Label131/LConn1 -- Seg 20/RConn3
  Connection Label130/LConn1 -- Seg 20/RConn2
  Connection Label19/LConn1 -- Seg 20/RConn1
  Connection Label129/LConn1 -- Seg 19/RConn3
  Connection Label128/LConn1 -- Seg 19/RConn2
  Connection Label18/LConn1 -- Seg 19/RConn1
  Connection Label127/LConn1 -- Seg 18/RConn3
  Connection Label126/LConn1 -- Seg 18/RConn2
  Connection Label17/LConn1 -- Seg 18/RConn1
  Connection Label125/LConn1 -- Seg 17/RConn3
  Connection Label124/LConn1 -- Seg 17/RConn2
  Connection Label16/LConn1 -- Seg 17/RConn1
  Connection Label123/LConn1 -- Seg 16/RConn3
  Connection Label122/LConn1 -- Seg 16/RConn2
  Connection Label15/LConn1 -- Seg 16/RConn1
  Connection Label121/LConn1 -- Seg 15/RConn3
  Connection Label120/LConn1 -- Seg 15/RConn2
  Connection Label14/LConn1 -- Seg 15/RConn1
  Connection Label119/LConn1 -- Seg 14/RConn3
  Connection Label118/LConn1 -- Seg 14/RConn2
  Connection Label13/LConn1 -- Seg 14/RConn1
  Connection Label117/LConn1 -- Seg 13/RConn3
  Connection Label116/LConn1 -- Seg 13/RConn2
  Connection Label12/LConn1 -- Seg 13/RConn1
  Connection Label115/LConn1 -- Seg 12/RConn3
  Connection Label114/LConn1 -- Seg 12/RConn2
  Connection Label11/LConn1 -- Seg 12/RConn1
  Connection Label113/LConn1 -- Seg 11/RConn3
  Connection Label112/LConn1 -- Seg 11/RConn2
  Connection Label10/LConn1 -- Seg 11/RConn1
  Connection Label111/LConn1 -- Seg 10/RConn3
  Connection Label110/LConn1 -- Seg 10/RConn2
  Connection Label9/LConn1 -- Seg 10/RConn1
  Connection Label109/LConn1 -- Seg 09/RConn3
  Connection Label108/LConn1 -- Seg 09/RConn2
  Connection Label8/LConn1 -- Seg 09/RConn1
  Connection Label107/LConn1 -- Seg 08/RConn3
  Connection Label106/LConn1 -- Seg 08/RConn2
  Connection Label7/LConn1 -- Seg 08/RConn1
  Connection Label105/LConn1 -- Seg 07/RConn3
  Connection Label104/LConn1 -- Seg 07/RConn2
  Connection Label6/LConn1 -- Seg 07/RConn1
  Connection Label103/LConn1 -- Seg 06/RConn3
  Connection Label102/LConn1 -- Seg 06/RConn2
  Connection Label5/LConn1 -- Seg 06/RConn1
  Connection Label101/LConn1 -- Seg 05/RConn3
  Connection Label100/LConn1 -- Seg 05/RConn2
  Connection Label4/LConn1 -- Seg 05/RConn1
  Connection Label99/LConn1 -- Seg 04/RConn3
  Connection Label98/LConn1 -- Seg 04/RConn2
  Connection Label3/LConn1 -- Seg 04/RConn1
  Connection Label97/LConn1 -- Seg 03/RConn3
  Connection Label96/LConn1 -- Seg 03/RConn2
  Connection Label2/LConn1 -- Seg 03/RConn1
  Connection Label95/LConn1 -- Seg 02/RConn3
  Connection Label94/LConn1 -- Seg 02/RConn2
  Connection Label1/LConn1 -- Seg 02/RConn1
  Connection Label93/LConn1 -- Seg 01/RConn3
  Connection Label92/LConn1 -- Seg 01/RConn2
  Connection Label/LConn1 -- Seg 01/RConn1
  Simscape Bus3/RConn1 -- T/RConn1
  Simscape Bus3/LConn9 -- Connection Label234/LConn1
  Simscape Bus3/LConn6 -- Connection Label231/LConn1
  Simscape Bus3/LConn11 -- Connection Label236/LConn1
  Simscape Bus3/LConn1 -- Connection Label272/LConn1
  Simscape Bus3/LConn2 -- Connection Label273/LConn1
  Simscape Bus3/LConn5 -- Connection Label230/LConn1
  Simscape Bus3/LConn7 -- Connection Label232/LConn1
  Simscape Bus3/LConn3 -- Connection Label274/LConn1
  Simscape Bus3/LConn23 -- Connection Label248/LConn1
  Simscape Bus3/LConn4 -- Connection Label275/LConn1
  Simscape Bus3/LConn8 -- Connection Label233/LConn1
  Simscape Bus3/LConn10 -- Connection Label235/LConn1
  Simscape Bus3/LConn12 -- Connection Label237/LConn1
  Simscape Bus3/LConn13 -- Connection Label238/LConn1
  Simscape Bus3/LConn14 -- Connection Label239/LConn1
  Simscape Bus3/LConn15 -- Connection Label240/LConn1
  Simscape Bus3/LConn16 -- Connection Label241/LConn1
  Simscape Bus3/LConn43 -- Connection Label268/LConn1
  Simscape Bus3/LConn17 -- Connection Label242/LConn1
  Simscape Bus3/LConn18 -- Connection Label243/LConn1
  Simscape Bus3/LConn19 -- Connection Label244/LConn1
  Simscape Bus3/LConn33 -- Connection Label258/LConn1
  Simscape Bus3/LConn20 -- Connection Label245/LConn1
  Simscape Bus3/LConn21 -- Connection Label246/LConn1
  Simscape Bus3/LConn38 -- Connection Label263/LConn1
  Simscape Bus3/LConn22 -- Connection Label247/LConn1
  Simscape Bus3/LConn24 -- Connection Label249/LConn1
  Simscape Bus3/LConn25 -- Connection Label250/LConn1
  Simscape Bus3/LConn26 -- Connection Label251/LConn1
  Simscape Bus3/LConn27 -- Connection Label252/LConn1
  Simscape Bus3/LConn28 -- Connection Label253/LConn1
  Simscape Bus3/LConn29 -- Connection Label254/LConn1
  Simscape Bus3/LConn30 -- Connection Label255/LConn1
  Simscape Bus3/LConn31 -- Connection Label256/LConn1
  Simscape Bus3/LConn32 -- Connection Label257/LConn1
  Simscape Bus3/LConn34 -- Connection Label259/LConn1
  Simscape Bus3/LConn35 -- Connection Label260/LConn1
  Simscape Bus3/LConn36 -- Connection Label261/LConn1
  Simscape Bus3/LConn45 -- Connection Label270/LConn1
  Simscape Bus3/LConn37 -- Connection Label262/LConn1
  Simscape Bus3/LConn39 -- Connection Label264/LConn1
  Simscape Bus3/LConn40 -- Connection Label265/LConn1
  Simscape Bus3/LConn41 -- Connection Label266/LConn1
  Simscape Bus3/LConn42 -- Connection Label267/LConn1
  Simscape Bus3/LConn44 -- Connection Label269/LConn1
  Simscape Bus3/LConn46 -- Connection Label271/LConn1
  Simscape Bus1/LConn46 -- Connection Label225/LConn1
  Simscape Bus1/LConn45 -- Connection Label224/LConn1
  Simscape Bus1/LConn44 -- Connection Label223/LConn1
  Simscape Bus1/LConn43 -- Connection Label222/LConn1
  Simscape Bus1/LConn42 -- Connection Label221/LConn1
  Simscape Bus1/LConn41 -- Connection Label220/LConn1
  Simscape Bus1/LConn40 -- Connection Label219/LConn1
  Simscape Bus1/LConn39 -- Connection Label218/LConn1
  Simscape Bus1/LConn38 -- Connection Label217/LConn1
  Simscape Bus1/LConn37 -- Connection Label216/LConn1
  Simscape Bus1/LConn36 -- Connection Label215/LConn1
  Simscape Bus1/LConn35 -- Connection Label214/LConn1
  Simscape Bus1/LConn34 -- Connection Label213/LConn1
  Simscape Bus1/LConn33 -- Connection Label212/LConn1
  Simscape Bus1/LConn32 -- Connection Label211/LConn1
  Simscape Bus1/LConn31 -- Connection Label210/LConn1
  Simscape Bus1/LConn30 -- Connection Label209/LConn1
  Simscape Bus1/LConn29 -- Connection Label208/LConn1
  Simscape Bus1/LConn28 -- Connection Label207/LConn1
  Simscape Bus1/LConn27 -- Connection Label206/LConn1
  Simscape Bus1/LConn26 -- Connection Label205/LConn1
  Simscape Bus1/LConn25 -- Connection Label204/LConn1
  Simscape Bus1/LConn24 -- Connection Label203/LConn1
  Simscape Bus1/LConn23 -- Connection Label202/LConn1
  Simscape Bus1/LConn22 -- Connection Label201/LConn1
  Simscape Bus1/LConn21 -- Connection Label200/LConn1
  Simscape Bus1/LConn20 -- Connection Label199/LConn1
  Simscape Bus1/LConn19 -- Connection Label198/LConn1
  Simscape Bus1/LConn18 -- Connection Label197/LConn1
  Simscape Bus1/LConn17 -- Connection Label196/LConn1
  Simscape Bus1/LConn16 -- Connection Label195/LConn1
  Simscape Bus1/LConn15 -- Connection Label194/LConn1
  Simscape Bus1/LConn14 -- Connection Label193/LConn1
  Simscape Bus1/LConn13 -- Connection Label192/LConn1
  Simscape Bus1/LConn12 -- Connection Label191/LConn1
  Simscape Bus1/LConn11 -- Connection Label190/LConn1
  Simscape Bus1/LConn10 -- Connection Label189/LConn1
  Simscape Bus1/LConn9 -- Connection Label188/LConn1
  Simscape Bus1/LConn8 -- Connection Label187/LConn1
  Simscape Bus1/LConn7 -- Connection Label186/LConn1
  Simscape Bus1/LConn6 -- Connection Label185/LConn1
  Simscape Bus1/LConn5 -- Connection Label184/LConn1
  Simscape Bus1/LConn4 -- Connection Label229/LConn1
  Simscape Bus1/LConn3 -- Connection Label228/LConn1
  Simscape Bus1/LConn2 -- Connection Label227/LConn1
  Simscape Bus1/LConn1 -- Connection Label226/LConn1
  Simscape Bus1/RConn1 -- G/RConn1
  R/RConn1 -- Simscape Bus2/RConn1
  Connection Label86/LConn1 -- Simscape Bus2/LConn46
  Connection Label85/LConn1 -- Simscape Bus2/LConn45
  Connection Label84/LConn1 -- Simscape Bus2/LConn44
  Connection Label83/LConn1 -- Simscape Bus2/LConn43
  Connection Label82/LConn1 -- Simscape Bus2/LConn42
  Connection Label81/LConn1 -- Simscape Bus2/LConn41
  Connection Label79/LConn1 -- Simscape Bus2/LConn40
  Connection Label78/LConn1 -- Simscape Bus2/LConn39
  Connection Label77/LConn1 -- Simscape Bus2/LConn38
  Connection Label76/LConn1 -- Simscape Bus2/LConn37
  Connection Label75/LConn1 -- Simscape Bus2/LConn36
  Connection Label74/LConn1 -- Simscape Bus2/LConn35
  Connection Label73/LConn1 -- Simscape Bus2/LConn34
  Connection Label72/LConn1 -- Simscape Bus2/LConn33
  Connection Label71/LConn1 -- Simscape Bus2/LConn32
  Connection Label70/LConn1 -- Simscape Bus2/LConn31
  Connection Label68/LConn1 -- Simscape Bus2/LConn30
  Connection Label67/LConn1 -- Simscape Bus2/LConn29
  Connection Label66/LConn1 -- Simscape Bus2/LConn28
  Connection Label65/LConn1 -- Simscape Bus2/LConn27
  Connection Label64/LConn1 -- Simscape Bus2/LConn26
  Connection Label63/LConn1 -- Simscape Bus2/LConn25
  Connection Label62/LConn1 -- Simscape Bus2/LConn24
  Connection Label61/LConn1 -- Simscape Bus2/LConn23
  Connection Label60/LConn1 -- Simscape Bus2/LConn22
  Connection Label59/LConn1 -- Simscape Bus2/LConn21
  Connection Label57/LConn1 -- Simscape Bus2/LConn20
  Connection Label56/LConn1 -- Simscape Bus2/LConn19
  Connection Label55/LConn1 -- Simscape Bus2/LConn18
  Connection Label54/LConn1 -- Simscape Bus2/LConn17
  Connection Label53/LConn1 -- Simscape Bus2/LConn16
  Connection Label52/LConn1 -- Simscape Bus2/LConn15
  Connection Label51/LConn1 -- Simscape Bus2/LConn14
  Connection Label50/LConn1 -- Simscape Bus2/LConn13
  Connection Label49/LConn1 -- Simscape Bus2/LConn12
  Connection Label48/LConn1 -- Simscape Bus2/LConn11
  Connection Label91/LConn1 -- Simscape Bus2/LConn10
  Connection Label90/LConn1 -- Simscape Bus2/LConn9
  Connection Label89/LConn1 -- Simscape Bus2/LConn8
  Connection Label88/LConn1 -- Simscape Bus2/LConn7
  Connection Label87/LConn1 -- Simscape Bus2/LConn6
  Connection Label80/LConn1 -- Simscape Bus2/LConn5
  Connection Label69/LConn1 -- Simscape Bus2/LConn4
  Connection Label58/LConn1 -- Simscape Bus2/LConn3
  Connection Label47/LConn1 -- Simscape Bus2/LConn2
  Connection Label46/LConn1 -- Simscape Bus2/LConn1
